simulink model "Antriebsstrangmodell_V1_4_n5"  (R2019a)
settings: Solver=FixedStepAuto  StartTime=0.0  StopTime=t_Simulation  FixedStep=dt  RelTol=1e-3
values from neighbouring files (symbols this model uses):
  A_Stirn = 2    [SIMULA~1.M]    (also in SIMULA~2.M)
  alpha_Luft = -4e-3    (= -0.004)    [SIMULA~1.M]    (also in SIMULA~2.M)
  alpha_Rotor = alpha_Al    (= 0.004)    [SIMULA~1.M]    (also in SIMULA~2.M)
  alpha_Stator = alpha_Al    (= 0.004)    [SIMULA~1.M]    (also in SIMULA~2.M)
  alpha_Ummag = -0.75e-3    (= -0.00075)    [SIMULA~1.M]    (also in SIMULA~2.M)
  c_W = 0.37    [SIMULA~1.M]    (also in SIMULA~2.M)
  COG_x = 1.4267    [SIMULA~1.M]    (also in SIMULA~2.M)
  COG_z = 0.4572    [SIMULA~1.M]    (also in SIMULA~2.M)
  cp_Luft = 1008.8    [SIMULA~1.M]    (also in SIMULA~2.M)
  e_Fahrzeug = 1.0478    [SIMULA~1.M]    (also in SIMULA~2.M)
  eta_EMaschine_Break_M_EMaschine = flipud(KennfeldMaschine.M(:,1))'    [SIMULA~1.M]    (also in SIMULA~2.M)
  eta_EMaschine_Break_M_EMaschine_reku = -KennfeldMaschine.M(:,1)'    [SIMULA~1.M]    (also in SIMULA~2.M)
  eta_EMaschine_Break_n_EMaschine = KennfeldMaschine.n(end-1,:)    [SIMULA~1.M]    (also in SIMULA~2.M)
  eta_EMaschine_Break_n_EMaschine_reku = KennfeldMaschine.n(end-1,:)    [SIMULA~1.M]    (also in SIMULA~2.M)
  eta_EMaschine_Faktor_Volllast = 0.98    [SIMULA~1.M]    (also in SIMULA~2.M)
  eta_EMaschine_Table = flip(KennfeldMaschine.etages,1)    [SIMULA~1.M]    (also in SIMULA~2.M)
  eta_EMaschine_Table_reku = KennfeldMaschine.etages    [SIMULA~1.M]    (also in SIMULA~2.M)
  eta_Getriebe = 0.96    [SIMULA~1.M]    (also in SIMULA~2.M)
  eta_IA = 0.5    [SIMULA~1.M]    (also in SIMULA~2.M)
  h_WC_pumpoff = Nu_WC*lam_WC/dh_WC    [SIMULA~1.M]    (also in SIMULA~2.M)
  h_WC_pumpon = Nu_WC*lam_WC/dh_WC    [SIMULA~1.M]    (also in SIMULA~2.M)
  i_Getriebe = 5.697    [SIMULA~1.M]    (also in SIMULA~2.M)
  krb_Korrektur = 0.53/10    (= 0.053)    [SIMULA~1.M]    (also in SIMULA~2.M)
  lam_Luft = 0.028592    [SIMULA~1.M]    (also in SIMULA~2.M)
  M_EMaschine_max = zeros(2,numel(eta_EMaschine_Break_n_EMaschine))    [SIMULA~1.M]    (also in SIMULA~2.M)
  m_Fahrzeug = 825    [SIMULA~1.M]    (also in SIMULA~2.M)
  m_Zuladung = 80    [SIMULA~1.M]    (also in SIMULA~2.M)
  nue_Luft = 19.230034390524e-6    (= 1.92300343905e-05)    [SIMULA~1.M]    (also in SIMULA~2.M)
  pump_start_limit = 273.15 + 33    (= 306.15)    [SIMULA~1.M]    (also in SIMULA~2.M)
  r_dynamisch = 0.2774    [SIMULA~1.M]    (also in SIMULA~2.M)
  rho_Luft = 1.2    [SIMULA~1.M]    (also in SIMULA~2.M)
  rho_Luft_EM = 1.0468    [SIMULA~1.M]    (also in SIMULA~2.M)
  share_EMaschine_Ummagnet_reku_Table = ser.gen.share_Ummagnetisierungsverluste    [SIMULA~1.M]    (also in SIMULA~2.M)
  share_EMaschine_Ummagnet_Table = ser.mot.share_Ummagnetisierungsverluste    [SIMULA~1.M]    (also in SIMULA~2.M)
  share_EMaschine_Wicklung_reku_Table = ser.gen.share_Wicklungsverluste    [SIMULA~1.M]    (also in SIMULA~2.M)
  share_EMaschine_Wicklung_Table = ser.mot.share_Wicklungsverluste    [SIMULA~1.M]    (also in SIMULA~2.M)
  share_EMaschine_WirkMech_reku_Table = ser.gen.share_WirkmechVerluste    [SIMULA~1.M]    (also in SIMULA~2.M)
  share_EMaschine_WirkMech_Table = ser.mot.share_WirkmechVerluste    [SIMULA~1.M]    (also in SIMULA~2.M)
  share_EMaschine_WirkZus_reku_Table = ser.gen.share_WirkZusVerl    [SIMULA~1.M]    (also in SIMULA~2.M)
  share_EMaschine_WirkZus_Table = ser.mot.share_WirkZusVerl    [SIMULA~1.M]    (also in SIMULA~2.M)
  T_Entwurf_Rotor = 273.15+20    (= 293.15)    [SIMULA~1.M]    (also in SIMULA~2.M)
  T_Entwurf_Stator = 273.15+20    (= 293.15)    [SIMULA~1.M]    (also in SIMULA~2.M)
  t_Simulation = v_Fahrzeug.Time(end)+1    [SIMULA~1.M]    (also in SIMULA~2.M = v_Fahrzeug.Time(end))
  T_Start_EMaschine = 273.15 + 23    (= 296.15)    [SIMULA~1.M]    (also in SIMULA~2.M)
  v_max = 110    [SIMULA~1.M]    (also in SIMULA~2.M)
  WB = 2.96    [SIMULA~1.M]    (also in SIMULA~2.M)
undefined symbols (not defined in the file or in its folder): A_AGP, A_IA, Anteil_Rotor_Ringe, Anteil_Stator, chi_Lager, D_2a, D_2r, delta, f_R, m_RTO, m_RYO, m_SSL_L, m_STO, m_SYO, m_WH_L, n_dis
libraries: fl_lib x440, nesl_utility x106, SimscapeCustomBlocks_lib x45, simulink x3
(part 2 of 5)

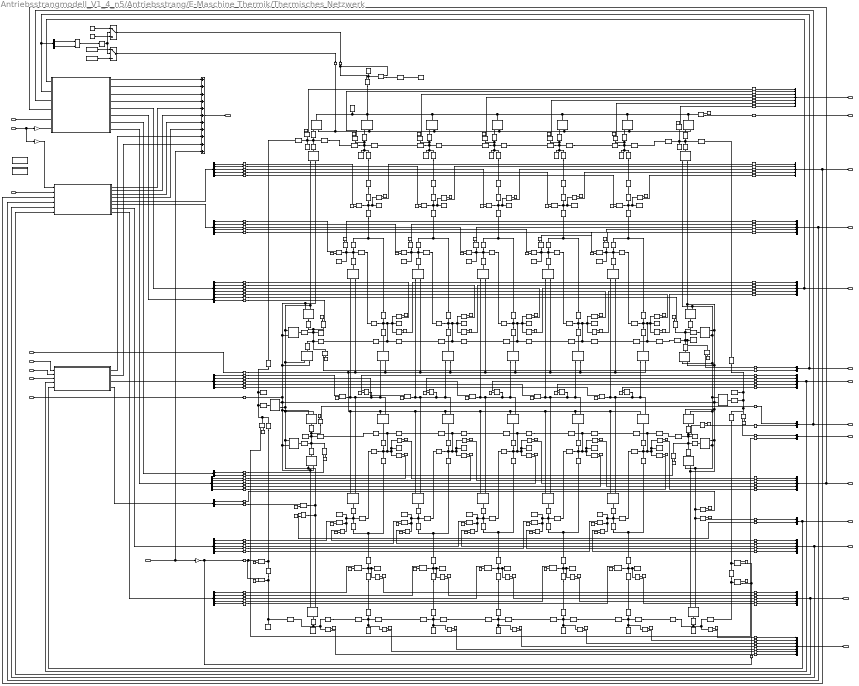
== system Antriebsstrangmodell_V1_4_n5/Antriebsstrang/E-Maschine Thermik/Thermisches Netzwerk ==
  note: Gehäusedeckel
  note: Gehäusedeckel
  note: Statorzähne
  note: Rotornuten
  note: Rotorwelle
  note: Lager
  note: Lager
  note: Rotorrücken
  note: Rotorzähne
  note: Kurzschluss-
      | ring
  note: Kurzschlussring
  note: Wickelkopf
  note: Wickelkopf
  note: Statornuten (Wicklung)
  note: Statorjoch
  note: Gehäuse
  P_EMaschine_Verlust_Wicklung [W] : Inport
  P_EMaschine_Verlust_Ummagnet [W] : Inport  Port=2
  P_EMaschine_Verlust_WirkZus [W] : Inport  Port=3
  P_EMaschine_Verlust_Lueftung [W] : Inport  Port=4
  P_EMaschine_Verlust_Lager [W] : Inport  Port=5
  HTC_Luftspalt [W*m^-2*K^-1] : Inport  Port=6
  HTC_fconv_Luftspalt [W*m^-2*K^-1] : Inport  Port=7
  HTC_Innenluft [W*m^-2*K^-1] : Inport  Port=8
  HTC_fconv_Innenluft [W*m^-2*K^-1] : Inport  Port=9
  Add : Sum  Inputs=+++++++++++
  Aufteilung + Temperaturabhängigkeit Lüftungsverluste : Subsystem
  Aufteilung + Temperaturabhängigkeit Ummagnetisierungsverluste : Subsystem
  Aufteilung Wicklungsverluste + Temperaturabhängiger ohmscher Widerstand : Subsystem
  Bus Creator{,1,3..7} (7 alike) : BusCreator  Inputs=5
  Bus Creator10 : BusCreator  Inputs=7
  Bus Creator11 : BusCreator  Inputs=7
  Bus Creator{2,8..9,12} (4 alike) : BusCreator  Inputs=2
  Bus Selector : BusSelector  OutputSignals=P_EMaschine_Verlust_SSL_1 [W],P_EMaschine_Verlust_SSL_2 [W],P_EMaschine_Verlust_SSL_3 [W],P_EMaschine_Verlust_SSL_4 [W],P_EMaschine_Verlust_SSL_5 [W]
  Bus Selector1 : BusSelector  OutputSignals=T_EMaschine_WH_2 [K],T_EMaschine_WH_1 [K]
  Bus Selector10 : BusSelector  OutputSignals=P_EMaschine_Verlust_IA_2 [W],P_EMaschine_Verlust_IA_1 [W]
  Bus Selector2 : BusSelector  OutputSignals=P_EMaschine_Verlust_WH_2 [W],P_EMaschine_Verlust_WH_1 [W]
  Bus Selector3 : BusSelector  OutputSignals=P_EMaschine_Verlust_ER_1 [W],P_EMaschine_Verlust_ER_2 [W]
  Bus Selector4 : BusSelector  OutputSignals=P_EMaschine_Verlust_RSL_1 [W],P_EMaschine_Verlust_RSL_2 [W],P_EMaschine_Verlust_RSL_3 [W],P_EMaschine_Verlust_RSL_4 [W],P_EMaschine_Verlust_RSL_5 [W]
  Bus Selector5 : BusSelector  OutputSignals=P_EMaschine_Verlust_AGP_1 [W],P_EMaschine_Verlust_AGP_2 [W],P_EMaschine_Verlust_AGP_3 [W],P_EMaschine_Verlust_AGP_4 [W],P_EMaschine_Verlust_AGP_5 [W]
  Bus Selector6 : BusSelector  OutputSignals=P_EMaschine_Verlust_STO_1 [W],P_EMaschine_Verlust_STO_2 [W],P_EMaschine_Verlust_STO_3 [W],P_EMaschine_Verlust_STO_4 [W],P_EMaschine_Verlust_STO_5 [W]
  Bus Selector7 : BusSelector  OutputSignals=P_EMaschine_Verlust_SYO_1 [W],P_EMaschine_Verlust_SYO_2 [W],P_EMaschine_Verlust_SYO_3 [W],P_EMaschine_Verlust_SYO_4 [W],P_EMaschine_Verlust_SYO_5 [W]
  Bus Selector8 : BusSelector  OutputSignals=P_EMaschine_Verlust_RTO_1 [W],P_EMaschine_Verlust_RTO_2 [W],P_EMaschine_Verlust_RTO_3 [W],P_EMaschine_Verlust_RTO_4 [W],P_EMaschine_Verlust_RTO_5 [W]
  Bus Selector9 : BusSelector  OutputSignals=P_EMaschine_Verlust_RYO_1 [W],P_EMaschine_Verlust_RYO_2 [W],P_EMaschine_Verlust_RYO_3 [W],P_EMaschine_Verlust_RYO_4 [W],P_EMaschine_Verlust_RYO_5 [W]
  C_EC(1) : fl_lib/Thermal/Thermal Elements/Thermal Mass  mass=m_EC kg  sp_heat=cp_EC J/kg/K  T_specify=on  T_priority=High  T=T_Start_EMaschine K  T_nominal_specify=off  T_nominal_unit=K  T_nominal_value=1  Q_specify=off  Q_priority=None  Q=0 W  Q_nominal_specify=off  Q_nominal_unit=W  Q_nominal_value=1
  C_EC(2) : fl_lib/Thermal/Thermal Elements/Thermal Mass  mass=m_EC kg  sp_heat=cp_EC J/kg/K  T_specify=on  T_priority=High  T=T_Start_EMaschine K  T_nominal_specify=off  T_nominal_unit=K  T_nominal_value=1  Q_specify=off  Q_priority=None  Q=0 W  Q_nominal_specify=off  Q_nominal_unit=W  Q_nominal_value=1
  C_ER(1) : fl_lib/Thermal/Thermal Elements/Thermal Mass  mass=m_ER kg  sp_heat=cp_ER J/kg/K  T_specify=on  T_priority=High  T=T_Start_EMaschine K  T_nominal_specify=off  T_nominal_unit=K  T_nominal_value=1  Q_specify=off  Q_priority=None  Q=0 W  Q_nominal_specify=off  Q_nominal_unit=W  Q_nominal_value=1
  C_ER(2) : fl_lib/Thermal/Thermal Elements/Thermal Mass  mass=m_ER kg  sp_heat=cp_ER J/kg/K  T_specify=on  T_priority=High  T=T_Start_EMaschine K  T_nominal_specify=off  T_nominal_unit=K  T_nominal_value=1  Q_specify=off  Q_priority=None  Q=0 W  Q_nominal_specify=off  Q_nominal_unit=W  Q_nominal_value=1
  C_HO_a(1) : fl_lib/Thermal/Thermal Elements/Thermal Mass  mass=m_HO_a kg  sp_heat=cp_HO J/kg/K  T_specify=on  T_priority=High  T=T_Start_EMaschine K  T_nominal_specify=off  T_nominal_unit=K  T_nominal_value=1  Q_specify=off  Q_priority=None  Q=0 W  Q_nominal_specify=off  Q_nominal_unit=W  Q_nominal_value=1
  C_HO_a(2) : fl_lib/Thermal/Thermal Elements/Thermal Mass  mass=m_HO_a kg  sp_heat=cp_HO J/kg/K  T_specify=on  T_priority=High  T=T_Start_EMaschine K  T_nominal_specify=off  T_nominal_unit=K  T_nominal_value=1  Q_specify=off  Q_priority=None  Q=0 W  Q_nominal_specify=off  Q_nominal_unit=W  Q_nominal_value=1
  C_HO_a(3) : fl_lib/Thermal/Thermal Elements/Thermal Mass  mass=m_HO_a kg  sp_heat=cp_HO J/kg/K  T_specify=on  T_priority=High  T=T_Start_EMaschine K  T_nominal_specify=off  T_nominal_unit=K  T_nominal_value=1  Q_specify=off  Q_priority=None  Q=0 W  Q_nominal_specify=off  Q_nominal_unit=W  Q_nominal_value=1
  C_HO_a(4) : fl_lib/Thermal/Thermal Elements/Thermal Mass  mass=m_HO_a kg  sp_heat=cp_HO J/kg/K  T_specify=on  T_priority=High  T=T_Start_EMaschine K  T_nominal_specify=off  T_nominal_unit=K  T_nominal_value=1  Q_specify=off  Q_priority=None  Q=0 W  Q_nominal_specify=off  Q_nominal_unit=W  Q_nominal_value=1
  C_HO_a(5) : fl_lib/Thermal/Thermal Elements/Thermal Mass  mass=m_HO_a kg  sp_heat=cp_HO J/kg/K  T_specify=on  T_priority=High  T=T_Start_EMaschine K  T_nominal_specify=off  T_nominal_unit=K  T_nominal_value=1  Q_specify=off  Q_priority=None  Q=0 W  Q_nominal_specify=off  Q_nominal_unit=W  Q_nominal_value=1
  C_HO_p(1) : fl_lib/Thermal/Thermal Elements/Thermal Mass  mass=m_HO_p kg  sp_heat=cp_HO J/kg/K  T_specify=on  T_priority=High  T=T_Start_EMaschine K  T_nominal_specify=off  T_nominal_unit=K  T_nominal_value=1  Q_specify=off  Q_priority=None  Q=0 W  Q_nominal_specify=off  Q_nominal_unit=W  Q_nominal_value=1
  C_HO_p(2) : fl_lib/Thermal/Thermal Elements/Thermal Mass  mass=m_HO_p kg  sp_heat=cp_HO J/kg/K  T_specify=on  T_priority=High  T=T_Start_EMaschine K  T_nominal_specify=off  T_nominal_unit=K  T_nominal_value=1  Q_specify=off  Q_priority=None  Q=0 W  Q_nominal_specify=off  Q_nominal_unit=W  Q_nominal_value=1
  C_RSL(1) : fl_lib/Thermal/Thermal Elements/Thermal Mass  mass=m_RSL kg  sp_heat=cp_RSL J/kg/K  T_specify=on  T_priority=High  T=T_Start_EMaschine K  T_nominal_specify=off  T_nominal_unit=K  T_nominal_value=1  Q_specify=off  Q_priority=None  Q=0 W  Q_nominal_specify=off  Q_nominal_unit=W  Q_nominal_value=1
  C_RSL(2) : fl_lib/Thermal/Thermal Elements/Thermal Mass  mass=m_RSL kg  sp_heat=cp_RSL J/kg/K  T_specify=on  T_priority=High  T=T_Start_EMaschine K  T_nominal_specify=off  T_nominal_unit=K  T_nominal_value=1  Q_specify=off  Q_priority=None  Q=0 W  Q_nominal_specify=off  Q_nominal_unit=W  Q_nominal_value=1
  C_RSL(3) : fl_lib/Thermal/Thermal Elements/Thermal Mass  mass=m_RSL kg  sp_heat=cp_RSL J/kg/K  T_specify=on  T_priority=High  T=T_Start_EMaschine K  T_nominal_specify=off  T_nominal_unit=K  T_nominal_value=1  Q_specify=off  Q_priority=None  Q=0 W  Q_nominal_specify=off  Q_nominal_unit=W  Q_nominal_value=1
  C_RSL(4) : fl_lib/Thermal/Thermal Elements/Thermal Mass  mass=m_RSL kg  sp_heat=cp_RSL J/kg/K  T_specify=on  T_priority=High  T=T_Start_EMaschine K  T_nominal_specify=off  T_nominal_unit=K  T_nominal_value=1  Q_specify=off  Q_priority=None  Q=0 W  Q_nominal_specify=off  Q_nominal_unit=W  Q_nominal_value=1
  C_RSL(5) : fl_lib/Thermal/Thermal Elements/Thermal Mass  mass=m_RSL kg  sp_heat=cp_RSL J/kg/K  T_specify=on  T_priority=High  T=T_Start_EMaschine K  T_nominal_specify=off  T_nominal_unit=K  T_nominal_value=1  Q_specify=off  Q_priority=None  Q=0 W  Q_nominal_specify=off  Q_nominal_unit=W  Q_nominal_value=1
  C_RTO(1) : fl_lib/Thermal/Thermal Elements/Thermal Mass  mass=m_RTO kg  sp_heat=cp_RTO J/kg/K  T_specify=on  T_priority=High  T=T_Start_EMaschine K  T_nominal_specify=off  T_nominal_unit=K  T_nominal_value=1  Q_specify=off  Q_priority=None  Q=0 W  Q_nominal_specify=off  Q_nominal_unit=W  Q_nominal_value=1
  C_RTO(2) : fl_lib/Thermal/Thermal Elements/Thermal Mass  mass=m_RTO kg  sp_heat=cp_RTO J/kg/K  T_specify=on  T_priority=High  T=T_Start_EMaschine K  T_nominal_specify=off  T_nominal_unit=K  T_nominal_value=1  Q_specify=off  Q_priority=None  Q=0 W  Q_nominal_specify=off  Q_nominal_unit=W  Q_nominal_value=1
  C_RTO(3) : fl_lib/Thermal/Thermal Elements/Thermal Mass  mass=m_RTO kg  sp_heat=cp_RTO J/kg/K  T_specify=on  T_priority=High  T=T_Start_EMaschine K  T_nominal_specify=off  T_nominal_unit=K  T_nominal_value=1  Q_specify=off  Q_priority=None  Q=0 W  Q_nominal_specify=off  Q_nominal_unit=W  Q_nominal_value=1
  C_RTO(4) : fl_lib/Thermal/Thermal Elements/Thermal Mass  mass=m_RTO kg  sp_heat=cp_RTO J/kg/K  T_specify=on  T_priority=High  T=T_Start_EMaschine K  T_nominal_specify=off  T_nominal_unit=K  T_nominal_value=1  Q_specify=off  Q_priority=None  Q=0 W  Q_nominal_specify=off  Q_nominal_unit=W  Q_nominal_value=1
  C_RTO(5) : fl_lib/Thermal/Thermal Elements/Thermal Mass  mass=m_RTO kg  sp_heat=cp_RTO J/kg/K  T_specify=on  T_priority=High  T=T_Start_EMaschine K  T_nominal_specify=off  T_nominal_unit=K  T_nominal_value=1  Q_specify=off  Q_priority=None  Q=0 W  Q_nominal_specify=off  Q_nominal_unit=W  Q_nominal_value=1
  C_RYO(1) : fl_lib/Thermal/Thermal Elements/Thermal Mass  mass=m_RYO kg  sp_heat=cp_RYO J/kg/K  T_specify=on  T_priority=High  T=T_Start_EMaschine K  T_nominal_specify=off  T_nominal_unit=K  T_nominal_value=1  Q_specify=off  Q_priority=None  Q=0 W  Q_nominal_specify=off  Q_nominal_unit=W  Q_nominal_value=1
  C_RYO(2) : fl_lib/Thermal/Thermal Elements/Thermal Mass  mass=m_RYO kg  sp_heat=cp_RYO J/kg/K  T_specify=on  T_priority=High  T=T_Start_EMaschine K  T_nominal_specify=off  T_nominal_unit=K  T_nominal_value=1  Q_specify=off  Q_priority=None  Q=0 W  Q_nominal_specify=off  Q_nominal_unit=W  Q_nominal_value=1
  C_RYO(3) : fl_lib/Thermal/Thermal Elements/Thermal Mass  mass=m_RYO kg  sp_heat=cp_RYO J/kg/K  T_specify=on  T_priority=High  T=T_Start_EMaschine K  T_nominal_specify=off  T_nominal_unit=K  T_nominal_value=1  Q_specify=off  Q_priority=None  Q=0 W  Q_nominal_specify=off  Q_nominal_unit=W  Q_nominal_value=1
  C_RYO(4) : fl_lib/Thermal/Thermal Elements/Thermal Mass  mass=m_RYO kg  sp_heat=cp_RYO J/kg/K  T_specify=on  T_priority=High  T=T_Start_EMaschine K  T_nominal_specify=off  T_nominal_unit=K  T_nominal_value=1  Q_specify=off  Q_priority=None  Q=0 W  Q_nominal_specify=off  Q_nominal_unit=W  Q_nominal_value=1
  C_RYO(5) : fl_lib/Thermal/Thermal Elements/Thermal Mass  mass=m_RYO kg  sp_heat=cp_RYO J/kg/K  T_specify=on  T_priority=High  T=T_Start_EMaschine K  T_nominal_specify=off  T_nominal_unit=K  T_nominal_value=1  Q_specify=off  Q_priority=None  Q=0 W  Q_nominal_specify=off  Q_nominal_unit=W  Q_nominal_value=1
  C_SH_a(1) : fl_lib/Thermal/Thermal Elements/Thermal Mass  mass=m_SH_a kg  sp_heat=cp_SH J/kg/K  T_specify=on  T_priority=High  T=T_Start_EMaschine K  T_nominal_specify=off  T_nominal_unit=K  T_nominal_value=1  Q_specify=off  Q_priority=None  Q=0 W  Q_nominal_specify=off  Q_nominal_unit=W  Q_nominal_value=1
  C_SH_a(2) : fl_lib/Thermal/Thermal Elements/Thermal Mass  mass=m_SH_a kg  sp_heat=cp_SH J/kg/K  T_specify=on  T_priority=High  T=T_Start_EMaschine K  T_nominal_specify=off  T_nominal_unit=K  T_nominal_value=1  Q_specify=off  Q_priority=None  Q=0 W  Q_nominal_specify=off  Q_nominal_unit=W  Q_nominal_value=1
  C_SH_a(3) : fl_lib/Thermal/Thermal Elements/Thermal Mass  mass=m_SH_a kg  sp_heat=cp_SH J/kg/K  T_specify=on  T_priority=High  T=T_Start_EMaschine K  T_nominal_specify=off  T_nominal_unit=K  T_nominal_value=1  Q_specify=off  Q_priority=None  Q=0 W  Q_nominal_specify=off  Q_nominal_unit=W  Q_nominal_value=1
  C_SH_a(4) : fl_lib/Thermal/Thermal Elements/Thermal Mass  mass=m_SH_a kg  sp_heat=cp_SH J/kg/K  T_specify=on  T_priority=High  T=T_Start_EMaschine K  T_nominal_specify=off  T_nominal_unit=K  T_nominal_value=1  Q_specify=off  Q_priority=None  Q=0 W  Q_nominal_specify=off  Q_nominal_unit=W  Q_nominal_value=1
  C_SH_a(5) : fl_lib/Thermal/Thermal Elements/Thermal Mass  mass=m_SH_a kg  sp_heat=cp_SH J/kg/K  T_specify=on  T_priority=High  T=T_Start_EMaschine K  T_nominal_specify=off  T_nominal_unit=K  T_nominal_value=1  Q_specify=off  Q_priority=None  Q=0 W  Q_nominal_specify=off  Q_nominal_unit=W  Q_nominal_value=1
  C_SH_p(1) : fl_lib/Thermal/Thermal Elements/Thermal Mass  mass=m_SH_p kg  sp_heat=cp_SH J/kg/K  T_specify=on  T_priority=High  T=T_Start_EMaschine K  T_nominal_specify=off  T_nominal_unit=K  T_nominal_value=1  Q_specify=off  Q_priority=None  Q=0 W  Q_nominal_specify=off  Q_nominal_unit=W  Q_nominal_value=1
  C_SH_p(2) : fl_lib/Thermal/Thermal Elements/Thermal Mass  mass=m_SH_p kg  sp_heat=cp_SH J/kg/K  T_specify=on  T_priority=High  T=T_Start_EMaschine K  T_nominal_specify=off  T_nominal_unit=K  T_nominal_value=1  Q_specify=off  Q_priority=None  Q=0 W  Q_nominal_specify=off  Q_nominal_unit=W  Q_nominal_value=1
  C_SSL(1) : fl_lib/Thermal/Thermal Elements/Thermal Mass  mass=m_SSL kg  sp_heat=cp_SSL J/kg/K  T_specify=on  T_priority=High  T=T_Start_EMaschine K  T_nominal_specify=off  T_nominal_unit=K  T_nominal_value=1  Q_specify=off  Q_priority=None  Q=0 W  Q_nominal_specify=off  Q_nominal_unit=W  Q_nominal_value=1
  C_SSL(2) : fl_lib/Thermal/Thermal Elements/Thermal Mass  mass=m_SSL kg  sp_heat=cp_SSL J/kg/K  T_specify=on  T_priority=High  T=T_Start_EMaschine K  T_nominal_specify=off  T_nominal_unit=K  T_nominal_value=1  Q_specify=off  Q_priority=None  Q=0 W  Q_nominal_specify=off  Q_nominal_unit=W  Q_nominal_value=1
  C_SSL(3) : fl_lib/Thermal/Thermal Elements/Thermal Mass  mass=m_SSL kg  sp_heat=cp_SSL J/kg/K  T_specify=on  T_priority=High  T=T_Start_EMaschine K  T_nominal_specify=off  T_nominal_unit=K  T_nominal_value=1  Q_specify=off  Q_priority=None  Q=0 W  Q_nominal_specify=off  Q_nominal_unit=W  Q_nominal_value=1
  C_SSL(4) : fl_lib/Thermal/Thermal Elements/Thermal Mass  mass=m_SSL kg  sp_heat=cp_SSL J/kg/K  T_specify=on  T_priority=High  T=T_Start_EMaschine K  T_nominal_specify=off  T_nominal_unit=K  T_nominal_value=1  Q_specify=off  Q_priority=None  Q=0 W  Q_nominal_specify=off  Q_nominal_unit=W  Q_nominal_value=1
  C_SSL(5) : fl_lib/Thermal/Thermal Elements/Thermal Mass  mass=m_SSL kg  sp_heat=cp_SSL J/kg/K  T_specify=on  T_priority=High  T=T_Start_EMaschine K  T_nominal_specify=off  T_nominal_unit=K  T_nominal_value=1  Q_specify=off  Q_priority=None  Q=0 W  Q_nominal_specify=off  Q_nominal_unit=W  Q_nominal_value=1
  C_STO(1) : fl_lib/Thermal/Thermal Elements/Thermal Mass  mass=m_STO kg  sp_heat=cp_STO J/kg/K  T_specify=on  T_priority=High  T=T_Start_EMaschine K  T_nominal_specify=off  T_nominal_unit=K  T_nominal_value=1  Q_specify=off  Q_priority=None  Q=0 W  Q_nominal_specify=off  Q_nominal_unit=W  Q_nominal_value=1
  C_STO(2) : fl_lib/Thermal/Thermal Elements/Thermal Mass  mass=m_STO kg  sp_heat=cp_STO J/kg/K  T_specify=on  T_priority=High  T=T_Start_EMaschine K  T_nominal_specify=off  T_nominal_unit=K  T_nominal_value=1  Q_specify=off  Q_priority=None  Q=0 W  Q_nominal_specify=off  Q_nominal_unit=W  Q_nominal_value=1
  C_STO(3) : fl_lib/Thermal/Thermal Elements/Thermal Mass  mass=m_STO kg  sp_heat=cp_STO J/kg/K  T_specify=on  T_priority=High  T=T_Start_EMaschine K  T_nominal_specify=off  T_nominal_unit=K  T_nominal_value=1  Q_specify=off  Q_priority=None  Q=0 W  Q_nominal_specify=off  Q_nominal_unit=W  Q_nominal_value=1
  C_STO(4) : fl_lib/Thermal/Thermal Elements/Thermal Mass  mass=m_STO kg  sp_heat=cp_STO J/kg/K  T_specify=on  T_priority=High  T=T_Start_EMaschine K  T_nominal_specify=off  T_nominal_unit=K  T_nominal_value=1  Q_specify=off  Q_priority=None  Q=0 W  Q_nominal_specify=off  Q_nominal_unit=W  Q_nominal_value=1
  C_STO(5) : fl_lib/Thermal/Thermal Elements/Thermal Mass  mass=m_STO kg  sp_heat=cp_STO J/kg/K  T_specify=on  T_priority=High  T=T_Start_EMaschine K  T_nominal_specify=off  T_nominal_unit=K  T_nominal_value=1  Q_specify=off  Q_priority=None  Q=0 W  Q_nominal_specify=off  Q_nominal_unit=W  Q_nominal_value=1
  C_SYO(1) : fl_lib/Thermal/Thermal Elements/Thermal Mass  mass=m_SYO kg  sp_heat=cp_SYO J/kg/K  T_specify=on  T_priority=High  T=T_Start_EMaschine K  T_nominal_specify=off  T_nominal_unit=K  T_nominal_value=1  Q_specify=off  Q_priority=None  Q=0 W  Q_nominal_specify=off  Q_nominal_unit=W  Q_nominal_value=1
  C_SYO(2) : fl_lib/Thermal/Thermal Elements/Thermal Mass  mass=m_SYO kg  sp_heat=cp_SYO J/kg/K  T_specify=on  T_priority=High  T=T_Start_EMaschine K  T_nominal_specify=off  T_nominal_unit=K  T_nominal_value=1  Q_specify=off  Q_priority=None  Q=0 W  Q_nominal_specify=off  Q_nominal_unit=W  Q_nominal_value=1
  C_SYO(3) : fl_lib/Thermal/Thermal Elements/Thermal Mass  mass=m_SYO kg  sp_heat=cp_SYO J/kg/K  T_specify=on  T_priority=High  T=T_Start_EMaschine K  T_nominal_specify=off  T_nominal_unit=K  T_nominal_value=1  Q_specify=off  Q_priority=None  Q=0 W  Q_nominal_specify=off  Q_nominal_unit=W  Q_nominal_value=1
  C_SYO(4) : fl_lib/Thermal/Thermal Elements/Thermal Mass  mass=m_SYO kg  sp_heat=cp_SYO J/kg/K  T_specify=on  T_priority=High  T=T_Start_EMaschine K  T_nominal_specify=off  T_nominal_unit=K  T_nominal_value=1  Q_specify=off  Q_priority=None  Q=0 W  Q_nominal_specify=off  Q_nominal_unit=W  Q_nominal_value=1
  C_SYO(5) : fl_lib/Thermal/Thermal Elements/Thermal Mass  mass=m_SYO kg  sp_heat=cp_SYO J/kg/K  T_specify=on  T_priority=High  T=T_Start_EMaschine K  T_nominal_specify=off  T_nominal_unit=K  T_nominal_value=1  Q_specify=off  Q_priority=None  Q=0 W  Q_nominal_specify=off  Q_nominal_unit=W  Q_nominal_value=1
  C_WC water cooling : fl_lib/Thermal/Thermal Elements/Thermal Mass  mass=m_WC kg  sp_heat=cp_WC J/kg/K  T_specify=on  T_priority=High  T=T_Start_EMaschine K  T_nominal_specify=off  T_nominal_unit=K  T_nominal_value=1  Q_specify=off  Q_priority=None  Q=0 W  Q_nominal_specify=off  Q_nominal_unit=W  Q_nominal_value=1
  C_WC water cooling pump active : fl_lib/Thermal/Thermal Elements/Thermal Mass  mass=m_WC_pumpon kg  sp_heat=cp_WC J/kg/K  T_specify=on  T_priority=High  T=T_Start_EMaschine K  T_nominal_specify=off  T_nominal_unit=K  T_nominal_value=1  Q_specify=off  Q_priority=None  Q=0 W  Q_nominal_specify=off  Q_nominal_unit=W  Q_nominal_value=1
  C_WH(1) : fl_lib/Thermal/Thermal Elements/Thermal Mass  mass=m_WH kg  sp_heat=cp_WH J/kg/K  T_specify=on  T_priority=High  T=T_Start_EMaschine K  T_nominal_specify=off  T_nominal_unit=K  T_nominal_value=1  Q_specify=off  Q_priority=None  Q=0 W  Q_nominal_specify=off  Q_nominal_unit=W  Q_nominal_value=1
  C_WH(2) : fl_lib/Thermal/Thermal Elements/Thermal Mass  mass=m_WH kg  sp_heat=cp_WH J/kg/K  T_specify=on  T_priority=High  T=T_Start_EMaschine K  T_nominal_specify=off  T_nominal_unit=K  T_nominal_value=1  Q_specify=off  Q_priority=None  Q=0 W  Q_nominal_specify=off  Q_nominal_unit=W  Q_nominal_value=1
  Convection HO to coolant (1) : SimscapeCustomBlocks_lib/Convective Heat Transfer  area=A_HO_p m^2  T_specify=off  T_priority=None  T=0 K  T_nominal_specify=off  T_nominal_unit=K  T_nominal_value=1  Q_specify=off  Q_priority=None  Q=0 W  Q_nominal_specify=off  Q_nominal_unit=W  Q_nominal_value=1
  Convection HO to coolant (2) : SimscapeCustomBlocks_lib/Convective Heat Transfer  area=A_HO_a m^2  T_specify=off  T_priority=None  T=0 K  T_nominal_specify=off  T_nominal_unit=K  T_nominal_value=1  Q_specify=off  Q_priority=None  Q=0 W  Q_nominal_specify=off  Q_nominal_unit=W  Q_nominal_value=1
  Convection HO to coolant (3) : SimscapeCustomBlocks_lib/Convective Heat Transfer  area=A_HO_a m^2  T_specify=off  T_priority=None  T=0 K  T_nominal_specify=off  T_nominal_unit=K  T_nominal_value=1  Q_specify=off  Q_priority=None  Q=0 W  Q_nominal_specify=off  Q_nominal_unit=W  Q_nominal_value=1
  Convection HO to coolant (4) : SimscapeCustomBlocks_lib/Convective Heat Transfer  area=A_HO_a m^2  T_specify=off  T_priority=None  T=0 K  T_nominal_specify=off  T_nominal_unit=K  T_nominal_value=1  Q_specify=off  Q_priority=None  Q=0 W  Q_nominal_specify=off  Q_nominal_unit=W  Q_nominal_value=1
  Convection HO to coolant (5) : SimscapeCustomBlocks_lib/Convective Heat Transfer  area=A_HO_a m^2  T_specify=off  T_priority=None  T=0 K  T_nominal_specify=off  T_nominal_unit=K  T_nominal_value=1  Q_specify=off  Q_priority=None  Q=0 W  Q_nominal_specify=off  Q_nominal_unit=W  Q_nominal_value=1
  Convection HO to coolant (6) : SimscapeCustomBlocks_lib/Convective Heat Transfer  area=A_HO_a m^2  T_specify=off  T_priority=None  T=0 K  T_nominal_specify=off  T_nominal_unit=K  T_nominal_value=1  Q_specify=off  Q_priority=None  Q=0 W  Q_nominal_specify=off  Q_nominal_unit=W  Q_nominal_value=1
  Convection HO to coolant (7) : SimscapeCustomBlocks_lib/Convective Heat Transfer  area=A_HO_p m^2  T_specify=off  T_priority=None  T=0 K  T_nominal_specify=off  T_nominal_unit=K  T_nominal_value=1  Q_specify=off  Q_priority=None  Q=0 W  Q_nominal_specify=off  Q_nominal_unit=W  Q_nominal_value=1
  Delay : Delay
  Gain4 : Gain  Gain=1/4
  HTC with coolant pump active : Constant  Value=h_WC_pumpon
  HTC with coolant pump inactive : Constant  Value=h_WC_pumpoff
  Konvektion Radiator an Umgebungsluft (keine Geschw.Abhängigkeit) : fl_lib/Thermal/Thermal Elements/Convective Heat Transfer  area=1 m^2  heat_tr_coeff=radiator_power W/(m^2 * K)  T_specify=off  T_priority=None  T=0 K  T_nominal_specify=off  T_nominal_unit=K  T_nominal_value=1  Q_specify=off  Q_priority=None  Q=0 W  Q_nominal_specify=off  Q_nominal_unit=W  Q_nominal_value=1
  MinMax : MinMax  Function=max  Inputs=2
  PS-Simulink Converter{1..58} (58 alike) : nesl_utility/PS-Simulink Converter  PhysicalDomain=network_engine_domain  SubClassName=ps_output  LeftPortType=input  RightPortType=output  PseudoPeriodic=off  Frequencies=[]  Unit=1  AffineConversion=off
  PV_AGP(1) : fl_lib/Thermal/Thermal Sources/Controlled Heat Flow Rate Source
      settings: SourceProductName=Simscape
  PV_AGP(2) : fl_lib/Thermal/Thermal Sources/Controlled Heat Flow Rate Source
      settings: SourceProductName=Simscape
  PV_AGP(3) : fl_lib/Thermal/Thermal Sources/Controlled Heat Flow Rate Source
      settings: SourceProductName=Simscape
  PV_AGP(4) : fl_lib/Thermal/Thermal Sources/Controlled Heat Flow Rate Source
      settings: SourceProductName=Simscape
  PV_AGP(5) : fl_lib/Thermal/Thermal Sources/Controlled Heat Flow Rate Source
      settings: SourceProductName=Simscape
  PV_BR(1.1) : fl_lib/Thermal/Thermal Sources/Controlled Heat Flow Rate Source
      settings: SourceProductName=Simscape
  PV_BR(1.2) : fl_lib/Thermal/Thermal Sources/Controlled Heat Flow Rate Source
      settings: SourceProductName=Simscape
  PV_BR(2.1) : fl_lib/Thermal/Thermal Sources/Controlled Heat Flow Rate Source
      settings: SourceProductName=Simscape
  PV_BR(2.2) : fl_lib/Thermal/Thermal Sources/Controlled Heat Flow Rate Source
      settings: SourceProductName=Simscape
  PV_ER(1) : fl_lib/Thermal/Thermal Sources/Controlled Heat Flow Rate Source
      settings: SourceProductName=Simscape
  PV_ER(2) : fl_lib/Thermal/Thermal Sources/Controlled Heat Flow Rate Source
      settings: SourceProductName=Simscape
  PV_IA(1) : fl_lib/Thermal/Thermal Sources/Controlled Heat Flow Rate Source
      settings: SourceProductName=Simscape
  PV_IA(2) : fl_lib/Thermal/Thermal Sources/Controlled Heat Flow Rate Source
      settings: SourceProductName=Simscape
  PV_RSL(1) : fl_lib/Thermal/Thermal Sources/Controlled Heat Flow Rate Source
      settings: SourceProductName=Simscape
  PV_RSL(2) : fl_lib/Thermal/Thermal Sources/Controlled Heat Flow Rate Source
      settings: SourceProductName=Simscape
  PV_RSL(3) : fl_lib/Thermal/Thermal Sources/Controlled Heat Flow Rate Source
      settings: SourceProductName=Simscape
  PV_RSL(4) : fl_lib/Thermal/Thermal Sources/Controlled Heat Flow Rate Source
      settings: SourceProductName=Simscape
  PV_RSL(5) : fl_lib/Thermal/Thermal Sources/Controlled Heat Flow Rate Source
      settings: SourceProductName=Simscape
  PV_RTO(1) : fl_lib/Thermal/Thermal Sources/Controlled Heat Flow Rate Source
      settings: SourceProductName=Simscape
  PV_RTO(2) : fl_lib/Thermal/Thermal Sources/Controlled Heat Flow Rate Source
      settings: SourceProductName=Simscape
  PV_RTO(3) : fl_lib/Thermal/Thermal Sources/Controlled Heat Flow Rate Source
      settings: SourceProductName=Simscape
  PV_RTO(4) : fl_lib/Thermal/Thermal Sources/Controlled Heat Flow Rate Source
      settings: SourceProductName=Simscape
  PV_RTO(5) : fl_lib/Thermal/Thermal Sources/Controlled Heat Flow Rate Source
      settings: SourceProductName=Simscape
  PV_RYO(1) : fl_lib/Thermal/Thermal Sources/Controlled Heat Flow Rate Source
      settings: SourceProductName=Simscape
  PV_RYO(2) : fl_lib/Thermal/Thermal Sources/Controlled Heat Flow Rate Source
      settings: SourceProductName=Simscape
  PV_RYO(3) : fl_lib/Thermal/Thermal Sources/Controlled Heat Flow Rate Source
      settings: SourceProductName=Simscape
  PV_RYO(4) : fl_lib/Thermal/Thermal Sources/Controlled Heat Flow Rate Source
      settings: SourceProductName=Simscape
  PV_RYO(5) : fl_lib/Thermal/Thermal Sources/Controlled Heat Flow Rate Source
      settings: SourceProductName=Simscape
  PV_SSL(1) : fl_lib/Thermal/Thermal Sources/Controlled Heat Flow Rate Source
      settings: SourceProductName=Simscape
  PV_SSL(2) : fl_lib/Thermal/Thermal Sources/Controlled Heat Flow Rate Source
      settings: SourceProductName=Simscape
  PV_SSL(3) : fl_lib/Thermal/Thermal Sources/Controlled Heat Flow Rate Source
      settings: SourceProductName=Simscape
  PV_SSL(4) : fl_lib/Thermal/Thermal Sources/Controlled Heat Flow Rate Source
      settings: SourceProductName=Simscape
  PV_SSL(5) : fl_lib/Thermal/Thermal Sources/Controlled Heat Flow Rate Source
      settings: SourceProductName=Simscape
  PV_STO(1) : fl_lib/Thermal/Thermal Sources/Controlled Heat Flow Rate Source
      settings: SourceProductName=Simscape
  PV_STO(2) : fl_lib/Thermal/Thermal Sources/Controlled Heat Flow Rate Source
      settings: SourceProductName=Simscape
  PV_STO(3) : fl_lib/Thermal/Thermal Sources/Controlled Heat Flow Rate Source
      settings: SourceProductName=Simscape
  PV_STO(4) : fl_lib/Thermal/Thermal Sources/Controlled Heat Flow Rate Source
      settings: SourceProductName=Simscape
  PV_STO(5) : fl_lib/Thermal/Thermal Sources/Controlled Heat Flow Rate Source
      settings: SourceProductName=Simscape
  PV_SYO(1) : fl_lib/Thermal/Thermal Sources/Controlled Heat Flow Rate Source
      settings: SourceProductName=Simscape
  PV_SYO(2) : fl_lib/Thermal/Thermal Sources/Controlled Heat Flow Rate Source
      settings: SourceProductName=Simscape
  PV_SYO(3) : fl_lib/Thermal/Thermal Sources/Controlled Heat Flow Rate Source
      settings: SourceProductName=Simscape
  PV_SYO(4) : fl_lib/Thermal/Thermal Sources/Controlled Heat Flow Rate Source
      settings: SourceProductName=Simscape
  PV_SYO(5) : fl_lib/Thermal/Thermal Sources/Controlled Heat Flow Rate Source
      settings: SourceProductName=Simscape
  PV_WH(1) : fl_lib/Thermal/Thermal Sources/Controlled Heat Flow Rate Source
      settings: SourceProductName=Simscape
  PV_WH(2) : fl_lib/Thermal/Thermal Sources/Controlled Heat Flow Rate Source
      settings: SourceProductName=Simscape
  R_contactBR(1) : fl_lib/Thermal/Thermal Elements/Thermal Resistance  resistance=R_contactBR K/W  T_specify=off  T_priority=None  T=0 K  T_nominal_specify=off  T_nominal_unit=K  T_nominal_value=1  Q_specify=off  Q_priority=None  Q=0 W  Q_nominal_specify=off  Q_nominal_unit=W  Q_nominal_value=1
      settings: SourceProductName=Simscape  SourceProductBaseCode=SS
  R_contactBR(2) : fl_lib/Thermal/Thermal Elements/Thermal Resistance  resistance=R_contactBR K/W  T_specify=off  T_priority=None  T=0 K  T_nominal_specify=off  T_nominal_unit=K  T_nominal_value=1  Q_specify=off  Q_priority=None  Q=0 W  Q_nominal_specify=off  Q_nominal_unit=W  Q_nominal_value=1
      settings: SourceProductName=Simscape  SourceProductBaseCode=SS
  R_contactHO (1) : fl_lib/Thermal/Thermal Elements/Thermal Resistance  resistance=R_contactHO K/W  T_specify=off  T_priority=None  T=0 K  T_nominal_specify=off  T_nominal_unit=K  T_nominal_value=1  Q_specify=off  Q_priority=None  Q=0 W  Q_nominal_specify=off  Q_nominal_unit=W  Q_nominal_value=1
      settings: SourceProductName=Simscape  SourceProductBaseCode=SS
  R_contactHO (2) : fl_lib/Thermal/Thermal Elements/Thermal Resistance  resistance=R_contactHO K/W  T_specify=off  T_priority=None  T=0 K  T_nominal_specify=off  T_nominal_unit=K  T_nominal_value=1  Q_specify=off  Q_priority=None  Q=0 W  Q_nominal_specify=off  Q_nominal_unit=W  Q_nominal_value=1
      settings: SourceProductName=Simscape  SourceProductBaseCode=SS
  R_contactHO (3) : fl_lib/Thermal/Thermal Elements/Thermal Resistance  resistance=R_contactHO K/W  T_specify=off  T_priority=None  T=0 K  T_nominal_specify=off  T_nominal_unit=K  T_nominal_value=1  Q_specify=off  Q_priority=None  Q=0 W  Q_nominal_specify=off  Q_nominal_unit=W  Q_nominal_value=1
      settings: SourceProductName=Simscape  SourceProductBaseCode=SS
  R_contactHO (4) : fl_lib/Thermal/Thermal Elements/Thermal Resistance  resistance=R_contactHO K/W  T_specify=off  T_priority=None  T=0 K  T_nominal_specify=off  T_nominal_unit=K  T_nominal_value=1  Q_specify=off  Q_priority=None  Q=0 W  Q_nominal_specify=off  Q_nominal_unit=W  Q_nominal_value=1
      settings: SourceProductName=Simscape  SourceProductBaseCode=SS
  R_contactHO (5) : fl_lib/Thermal/Thermal Elements/Thermal Resistance  resistance=R_contactHO K/W  T_specify=off  T_priority=None  T=0 K  T_nominal_specify=off  T_nominal_unit=K  T_nominal_value=1  Q_specify=off  Q_priority=None  Q=0 W  Q_nominal_specify=off  Q_nominal_unit=W  Q_nominal_value=1
      settings: SourceProductName=Simscape  SourceProductBaseCode=SS
  R_toBR2(1) : fl_lib/Thermal/Thermal Elements/Thermal Resistance  resistance=R_toBR2 K/W  T_specify=off  T_priority=None  T=0 K  T_nominal_specify=off  T_nominal_unit=K  T_nominal_value=1  Q_specify=off  Q_priority=None  Q=0 W  Q_nominal_specify=off  Q_nominal_unit=W  Q_nominal_value=1
      settings: SourceProductName=Simscape  SourceProductBaseCode=SS
  R_toBR2(2) : fl_lib/Thermal/Thermal Elements/Thermal Resistance  resistance=R_toBR2 K/W  T_specify=off  T_priority=None  T=0 K  T_nominal_specify=off  T_nominal_unit=K  T_nominal_value=1  Q_specify=off  Q_priority=None  Q=0 W  Q_nominal_specify=off  Q_nominal_unit=W  Q_nominal_value=1
      settings: SourceProductName=Simscape  SourceProductBaseCode=SS
  R_toBR_a(1.1) : fl_lib/Thermal/Thermal Elements/Thermal Resistance  resistance=R_toBR_a K/W  T_specify=off  T_priority=None  T=0 K  T_nominal_specify=off  T_nominal_unit=K  T_nominal_value=1  Q_specify=off  Q_priority=None  Q=0 W  Q_nominal_specify=off  Q_nominal_unit=W  Q_nominal_value=1
      settings: SourceProductName=Simscape  SourceProductBaseCode=SS
  R_toBR_a(1.2) : fl_lib/Thermal/Thermal Elements/Thermal Resistance  resistance=R_toBR_a K/W  T_specify=off  T_priority=None  T=0 K  T_nominal_specify=off  T_nominal_unit=K  T_nominal_value=1  Q_specify=off  Q_priority=None  Q=0 W  Q_nominal_specify=off  Q_nominal_unit=W  Q_nominal_value=1
      settings: SourceProductName=Simscape  SourceProductBaseCode=SS
  R_toBR_a(2.1) : fl_lib/Thermal/Thermal Elements/Thermal Resistance  resistance=R_toBR_a K/W  T_specify=off  T_priority=None  T=0 K  T_nominal_specify=off  T_nominal_unit=K  T_nominal_value=1  Q_specify=off  Q_priority=None  Q=0 W  Q_nominal_specify=off  Q_nominal_unit=W  Q_nominal_value=1
      settings: SourceProductName=Simscape  SourceProductBaseCode=SS
  R_toBR_a(2.2) : fl_lib/Thermal/Thermal Elements/Thermal Resistance  resistance=R_toBR_a K/W  T_specify=off  T_priority=None  T=0 K  T_nominal_specify=off  T_nominal_unit=K  T_nominal_value=1  Q_specify=off  Q_priority=None  Q=0 W  Q_nominal_specify=off  Q_nominal_unit=W  Q_nominal_value=1
      settings: SourceProductName=Simscape  SourceProductBaseCode=SS
  R_toBR_a(3.1) : fl_lib/Thermal/Thermal Elements/Thermal Resistance  resistance=R_toBR_a K/W  T_specify=off  T_priority=None  T=0 K  T_nominal_specify=off  T_nominal_unit=K  T_nominal_value=1  Q_specify=off  Q_priority=None  Q=0 W  Q_nominal_specify=off  Q_nominal_unit=W  Q_nominal_value=1
      settings: SourceProductName=Simscape  SourceProductBaseCode=SS
  R_toBR_a(3.2) : fl_lib/Thermal/Thermal Elements/Thermal Resistance  resistance=R_toBR_a K/W  T_specify=off  T_priority=None  T=0 K  T_nominal_specify=off  T_nominal_unit=K  T_nominal_value=1  Q_specify=off  Q_priority=None  Q=0 W  Q_nominal_specify=off  Q_nominal_unit=W  Q_nominal_value=1
      settings: SourceProductName=Simscape  SourceProductBaseCode=SS
  R_toBR_a(4.1) : fl_lib/Thermal/Thermal Elements/Thermal Resistance  resistance=R_toBR_a K/W  T_specify=off  T_priority=None  T=0 K  T_nominal_specify=off  T_nominal_unit=K  T_nominal_value=1  Q_specify=off  Q_priority=None  Q=0 W  Q_nominal_specify=off  Q_nominal_unit=W  Q_nominal_value=1
      settings: SourceProductName=Simscape  SourceProductBaseCode=SS
  R_toBR_a(4.2) : fl_lib/Thermal/Thermal Elements/Thermal Resistance  resistance=R_toBR_a K/W  T_specify=off  T_priority=None  T=0 K  T_nominal_specify=off  T_nominal_unit=K  T_nominal_value=1  Q_specify=off  Q_priority=None  Q=0 W  Q_nominal_specify=off  Q_nominal_unit=W  Q_nominal_value=1
      settings: SourceProductName=Simscape  SourceProductBaseCode=SS
  R_toBR_a(5.1) : fl_lib/Thermal/Thermal Elements/Thermal Resistance  resistance=R_toBR_a K/W  T_specify=off  T_priority=None  T=0 K  T_nominal_specify=off  T_nominal_unit=K  T_nominal_value=1  Q_specify=off  Q_priority=None  Q=0 W  Q_nominal_specify=off  Q_nominal_unit=W  Q_nominal_value=1
      settings: SourceProductName=Simscape  SourceProductBaseCode=SS
  R_toBR_a(5.2) : fl_lib/Thermal/Thermal Elements/Thermal Resistance  resistance=R_toBR_a K/W  T_specify=off  T_priority=None  T=0 K  T_nominal_specify=off  T_nominal_unit=K  T_nominal_value=1  Q_specify=off  Q_priority=None  Q=0 W  Q_nominal_specify=off  Q_nominal_unit=W  Q_nominal_value=1
      settings: SourceProductName=Simscape  SourceProductBaseCode=SS
  R_toBR_p(1.1) : fl_lib/Thermal/Thermal Elements/Thermal Resistance  resistance=R_toBR_p K/W  T_specify=off  T_priority=None  T=0 K  T_nominal_specify=off  T_nominal_unit=K  T_nominal_value=1  Q_specify=off  Q_priority=None  Q=0 W  Q_nominal_specify=off  Q_nominal_unit=W  Q_nominal_value=1
      settings: SourceProductName=Simscape  SourceProductBaseCode=SS
  R_toBR_p(1.2) : fl_lib/Thermal/Thermal Elements/Thermal Resistance  resistance=R_toBR_p K/W  T_specify=off  T_priority=None  T=0 K  T_nominal_specify=off  T_nominal_unit=K  T_nominal_value=1  Q_specify=off  Q_priority=None  Q=0 W  Q_nominal_specify=off  Q_nominal_unit=W  Q_nominal_value=1
      settings: SourceProductName=Simscape  SourceProductBaseCode=SS
  R_toBR_p(2.1) : fl_lib/Thermal/Thermal Elements/Thermal Resistance  resistance=R_toBR_p K/W  T_specify=off  T_priority=None  T=0 K  T_nominal_specify=off  T_nominal_unit=K  T_nominal_value=1  Q_specify=off  Q_priority=None  Q=0 W  Q_nominal_specify=off  Q_nominal_unit=W  Q_nominal_value=1
      settings: SourceProductName=Simscape  SourceProductBaseCode=SS
  R_toBR_p(2.2) : fl_lib/Thermal/Thermal Elements/Thermal Resistance  resistance=R_toBR_p K/W  T_specify=off  T_priority=None  T=0 K  T_nominal_specify=off  T_nominal_unit=K  T_nominal_value=1  Q_specify=off  Q_priority=None  Q=0 W  Q_nominal_specify=off  Q_nominal_unit=W  Q_nominal_value=1
      settings: SourceProductName=Simscape  SourceProductBaseCode=SS
  R_toEC_a(1.1) : fl_lib/Thermal/Thermal Elements/Thermal Resistance  resistance=R_toEC_a K/W  T_specify=off  T_priority=None  T=0 K  T_nominal_specify=off  T_nominal_unit=K  T_nominal_value=1  Q_specify=off  Q_priority=None  Q=0 W  Q_nominal_specify=off  Q_nominal_unit=W  Q_nominal_value=1
      settings: SourceProductName=Simscape  SourceProductBaseCode=SS
  R_toEC_a(1.2) : fl_lib/Thermal/Thermal Elements/Thermal Resistance  resistance=R_toEC_a K/W  T_specify=off  T_priority=None  T=0 K  T_nominal_specify=off  T_nominal_unit=K  T_nominal_value=1  Q_specify=off  Q_priority=None  Q=0 W  Q_nominal_specify=off  Q_nominal_unit=W  Q_nominal_value=1
      settings: SourceProductName=Simscape  SourceProductBaseCode=SS
  R_toEC_a(2.1) : fl_lib/Thermal/Thermal Elements/Thermal Resistance  resistance=R_toEC_a K/W  T_specify=off  T_priority=None  T=0 K  T_nominal_specify=off  T_nominal_unit=K  T_nominal_value=1  Q_specify=off  Q_priority=None  Q=0 W  Q_nominal_specify=off  Q_nominal_unit=W  Q_nominal_value=1
      settings: SourceProductName=Simscape  SourceProductBaseCode=SS
  R_toEC_a(2.2) : fl_lib/Thermal/Thermal Elements/Thermal Resistance  resistance=R_toEC_a K/W  T_specify=off  T_priority=None  T=0 K  T_nominal_specify=off  T_nominal_unit=K  T_nominal_value=1  Q_specify=off  Q_priority=None  Q=0 W  Q_nominal_specify=off  Q_nominal_unit=W  Q_nominal_value=1
      settings: SourceProductName=Simscape  SourceProductBaseCode=SS
  R_toEC_a(3.1) : fl_lib/Thermal/Thermal Elements/Thermal Resistance  resistance=R_toEC_a K/W  T_specify=off  T_priority=None  T=0 K  T_nominal_specify=off  T_nominal_unit=K  T_nominal_value=1  Q_specify=off  Q_priority=None  Q=0 W  Q_nominal_specify=off  Q_nominal_unit=W  Q_nominal_value=1
      settings: SourceProductName=Simscape  SourceProductBaseCode=SS
  R_toEC_a(3.2) : fl_lib/Thermal/Thermal Elements/Thermal Resistance  resistance=R_toEC_a K/W  T_specify=off  T_priority=None  T=0 K  T_nominal_specify=off  T_nominal_unit=K  T_nominal_value=1  Q_specify=off  Q_priority=None  Q=0 W  Q_nominal_specify=off  Q_nominal_unit=W  Q_nominal_value=1
      settings: SourceProductName=Simscape  SourceProductBaseCode=SS
  R_toEC_a(4.1) : fl_lib/Thermal/Thermal Elements/Thermal Resistance  resistance=R_toEC_a K/W  T_specify=off  T_priority=None  T=0 K  T_nominal_specify=off  T_nominal_unit=K  T_nominal_value=1  Q_specify=off  Q_priority=None  Q=0 W  Q_nominal_specify=off  Q_nominal_unit=W  Q_nominal_value=1
      settings: SourceProductName=Simscape  SourceProductBaseCode=SS
  R_toEC_a(4.2) : fl_lib/Thermal/Thermal Elements/Thermal Resistance  resistance=R_toEC_a K/W  T_specify=off  T_priority=None  T=0 K  T_nominal_specify=off  T_nominal_unit=K  T_nominal_value=1  Q_specify=off  Q_priority=None  Q=0 W  Q_nominal_specify=off  Q_nominal_unit=W  Q_nominal_value=1
      settings: SourceProductName=Simscape  SourceProductBaseCode=SS
  R_toEC_a(5.1) : fl_lib/Thermal/Thermal Elements/Thermal Resistance  resistance=R_toEC_a K/W  T_specify=off  T_priority=None  T=0 K  T_nominal_specify=off  T_nominal_unit=K  T_nominal_value=1  Q_specify=off  Q_priority=None  Q=0 W  Q_nominal_specify=off  Q_nominal_unit=W  Q_nominal_value=1
      settings: SourceProductName=Simscape  SourceProductBaseCode=SS
  R_toEC_a(5.2) : fl_lib/Thermal/Thermal Elements/Thermal Resistance  resistance=R_toEC_a K/W  T_specify=off  T_priority=None  T=0 K  T_nominal_specify=off  T_nominal_unit=K  T_nominal_value=1  Q_specify=off  Q_priority=None  Q=0 W  Q_nominal_specify=off  Q_nominal_unit=W  Q_nominal_value=1
      settings: SourceProductName=Simscape  SourceProductBaseCode=SS
  R_toEC_p(1.1) : fl_lib/Thermal/Thermal Elements/Thermal Resistance  resistance=R_toEC_p K/W  T_specify=off  T_priority=None  T=0 K  T_nominal_specify=off  T_nominal_unit=K  T_nominal_value=1  Q_specify=off  Q_priority=None  Q=0 W  Q_nominal_specify=off  Q_nominal_unit=W  Q_nominal_value=1
      settings: SourceProductName=Simscape  SourceProductBaseCode=SS
  R_toEC_p(1.2) : fl_lib/Thermal/Thermal Elements/Thermal Resistance  resistance=R_toEC_p K/W  T_specify=off  T_priority=None  T=0 K  T_nominal_specify=off  T_nominal_unit=K  T_nominal_value=1  Q_specify=off  Q_priority=None  Q=0 W  Q_nominal_specify=off  Q_nominal_unit=W  Q_nominal_value=1
      settings: SourceProductName=Simscape  SourceProductBaseCode=SS
  R_toEC_p(2.1) : fl_lib/Thermal/Thermal Elements/Thermal Resistance  resistance=R_toEC_p K/W  T_specify=off  T_priority=None  T=0 K  T_nominal_specify=off  T_nominal_unit=K  T_nominal_value=1  Q_specify=off  Q_priority=None  Q=0 W  Q_nominal_specify=off  Q_nominal_unit=W  Q_nominal_value=1
      settings: SourceProductName=Simscape  SourceProductBaseCode=SS
  R_toEC_p(2.2) : fl_lib/Thermal/Thermal Elements/Thermal Resistance  resistance=R_toEC_p K/W  T_specify=off  T_priority=None  T=0 K  T_nominal_specify=off  T_nominal_unit=K  T_nominal_value=1  Q_specify=off  Q_priority=None  Q=0 W  Q_nominal_specify=off  Q_nominal_unit=W  Q_nominal_value=1
      settings: SourceProductName=Simscape  SourceProductBaseCode=SS
  R_toER(1.1) : fl_lib/Thermal/Thermal Elements/Thermal Resistance  resistance=R_toER K/W  T_specify=off  T_priority=None  T=0 K  T_nominal_specify=off  T_nominal_unit=K  T_nominal_value=1  Q_specify=off  Q_priority=None  Q=0 W  Q_nominal_specify=off  Q_nominal_unit=W  Q_nominal_value=1
      settings: SourceProductName=Simscape  SourceProductBaseCode=SS
  R_toER(1.2) : fl_lib/Thermal/Thermal Elements/Thermal Resistance  resistance=R_toER K/W  T_specify=off  T_priority=None  T=0 K  T_nominal_specify=off  T_nominal_unit=K  T_nominal_value=1  Q_specify=off  Q_priority=None  Q=0 W  Q_nominal_specify=off  Q_nominal_unit=W  Q_nominal_value=1
      settings: SourceProductName=Simscape  SourceProductBaseCode=SS
  R_toER(2.1) : fl_lib/Thermal/Thermal Elements/Thermal Resistance  resistance=R_toER K/W  T_specify=off  T_priority=None  T=0 K  T_nominal_specify=off  T_nominal_unit=K  T_nominal_value=1  Q_specify=off  Q_priority=None  Q=0 W  Q_nominal_specify=off  Q_nominal_unit=W  Q_nominal_value=1
      settings: SourceProductName=Simscape  SourceProductBaseCode=SS
  R_toER(2.2) : fl_lib/Thermal/Thermal Elements/Thermal Resistance  resistance=R_toER K/W  T_specify=off  T_priority=None  T=0 K  T_nominal_specify=off  T_nominal_unit=K  T_nominal_value=1  Q_specify=off  Q_priority=None  Q=0 W  Q_nominal_specify=off  Q_nominal_unit=W  Q_nominal_value=1
      settings: SourceProductName=Simscape  SourceProductBaseCode=SS
  R_toER(3.1) : fl_lib/Thermal/Thermal Elements/Thermal Resistance  resistance=R_toER K/W  T_specify=off  T_priority=None  T=0 K  T_nominal_specify=off  T_nominal_unit=K  T_nominal_value=1  Q_specify=off  Q_priority=None  Q=0 W  Q_nominal_specify=off  Q_nominal_unit=W  Q_nominal_value=1
      settings: SourceProductName=Simscape  SourceProductBaseCode=SS
  R_toER(3.2) : fl_lib/Thermal/Thermal Elements/Thermal Resistance  resistance=R_toER K/W  T_specify=off  T_priority=None  T=0 K  T_nominal_specify=off  T_nominal_unit=K  T_nominal_value=1  Q_specify=off  Q_priority=None  Q=0 W  Q_nominal_specify=off  Q_nominal_unit=W  Q_nominal_value=1
      settings: SourceProductName=Simscape  SourceProductBaseCode=SS
  R_toER(4.1) : fl_lib/Thermal/Thermal Elements/Thermal Resistance  resistance=R_toER K/W  T_specify=off  T_priority=None  T=0 K  T_nominal_specify=off  T_nominal_unit=K  T_nominal_value=1  Q_specify=off  Q_priority=None  Q=0 W  Q_nominal_specify=off  Q_nominal_unit=W  Q_nominal_value=1
      settings: SourceProductName=Simscape  SourceProductBaseCode=SS
  R_toER(4.2) : fl_lib/Thermal/Thermal Elements/Thermal Resistance  resistance=R_toER K/W  T_specify=off  T_priority=None  T=0 K  T_nominal_specify=off  T_nominal_unit=K  T_nominal_value=1  Q_specify=off  Q_priority=None  Q=0 W  Q_nominal_specify=off  Q_nominal_unit=W  Q_nominal_value=1
      settings: SourceProductName=Simscape  SourceProductBaseCode=SS
  R_toER(5.1) : fl_lib/Thermal/Thermal Elements/Thermal Resistance  resistance=R_toER K/W  T_specify=off  T_priority=None  T=0 K  T_nominal_specify=off  T_nominal_unit=K  T_nominal_value=1  Q_specify=off  Q_priority=None  Q=0 W  Q_nominal_specify=off  Q_nominal_unit=W  Q_nominal_value=1
      settings: SourceProductName=Simscape  SourceProductBaseCode=SS
  R_toER(5.2) : fl_lib/Thermal/Thermal Elements/Thermal Resistance  resistance=R_toER K/W  T_specify=off  T_priority=None  T=0 K  T_nominal_specify=off  T_nominal_unit=K  T_nominal_value=1  Q_specify=off  Q_priority=None  Q=0 W  Q_nominal_specify=off  Q_nominal_unit=W  Q_nominal_value=1
      settings: SourceProductName=Simscape  SourceProductBaseCode=SS
  R_toHO(1) : fl_lib/Thermal/Thermal Elements/Thermal Resistance  resistance=R_toHO K/W  T_specify=off  T_priority=None  T=0 K  T_nominal_specify=off  T_nominal_unit=K  T_nominal_value=1  Q_specify=off  Q_priority=None  Q=0 W  Q_nominal_specify=off  Q_nominal_unit=W  Q_nominal_value=1
      settings: SourceProductName=Simscape  SourceProductBaseCode=SS
  R_toHO(2) : fl_lib/Thermal/Thermal Elements/Thermal Resistance  resistance=R_toHO K/W  T_specify=off  T_priority=None  T=0 K  T_nominal_specify=off  T_nominal_unit=K  T_nominal_value=1  Q_specify=off  Q_priority=None  Q=0 W  Q_nominal_specify=off  Q_nominal_unit=W  Q_nominal_value=1
      settings: SourceProductName=Simscape  SourceProductBaseCode=SS
  R_toHO(3) : fl_lib/Thermal/Thermal Elements/Thermal Resistance  resistance=R_toHO K/W  T_specify=off  T_priority=None  T=0 K  T_nominal_specify=off  T_nominal_unit=K  T_nominal_value=1  Q_specify=off  Q_priority=None  Q=0 W  Q_nominal_specify=off  Q_nominal_unit=W  Q_nominal_value=1
      settings: SourceProductName=Simscape  SourceProductBaseCode=SS
  R_toHO(4) : fl_lib/Thermal/Thermal Elements/Thermal Resistance  resistance=R_toHO K/W  T_specify=off  T_priority=None  T=0 K  T_nominal_specify=off  T_nominal_unit=K  T_nominal_value=1  Q_specify=off  Q_priority=None  Q=0 W  Q_nominal_specify=off  Q_nominal_unit=W  Q_nominal_value=1
      settings: SourceProductName=Simscape  SourceProductBaseCode=SS
  R_toHO(5) : fl_lib/Thermal/Thermal Elements/Thermal Resistance  resistance=R_toHO K/W  T_specify=off  T_priority=None  T=0 K  T_nominal_specify=off  T_nominal_unit=K  T_nominal_value=1  Q_specify=off  Q_priority=None  Q=0 W  Q_nominal_specify=off  Q_nominal_unit=W  Q_nominal_value=1
      settings: SourceProductName=Simscape  SourceProductBaseCode=SS
  R_toHO2(1) : fl_lib/Thermal/Thermal Elements/Thermal Resistance  resistance=R_toHO2 K/W  T_specify=off  T_priority=None  T=0 K  T_nominal_specify=off  T_nominal_unit=K  T_nominal_value=1  Q_specify=off  Q_priority=None  Q=0 W  Q_nominal_specify=off  Q_nominal_unit=W  Q_nominal_value=1
      settings: SourceProductName=Simscape  SourceProductBaseCode=SS
  R_toHO2(2) : fl_lib/Thermal/Thermal Elements/Thermal Resistance  resistance=R_toHO2 K/W  T_specify=off  T_priority=None  T=0 K  T_nominal_specify=off  T_nominal_unit=K  T_nominal_value=1  Q_specify=off  Q_priority=None  Q=0 W  Q_nominal_specify=off  Q_nominal_unit=W  Q_nominal_value=1
      settings: SourceProductName=Simscape  SourceProductBaseCode=SS
  R_toIA(1) : fl_lib/Thermal/Thermal Elements/Thermal Resistance  resistance=R_toIA K/W  T_specify=off  T_priority=None  T=0 K  T_nominal_specify=off  T_nominal_unit=K  T_nominal_value=1  Q_specify=off  Q_priority=None  Q=0 W  Q_nominal_specify=off  Q_nominal_unit=W  Q_nominal_value=1
      settings: SourceProductName=Simscape  SourceProductBaseCode=SS
  R_toIA(2) : fl_lib/Thermal/Thermal Elements/Thermal Resistance  resistance=R_toIA K/W  T_specify=off  T_priority=None  T=0 K  T_nominal_specify=off  T_nominal_unit=K  T_nominal_value=1  Q_specify=off  Q_priority=None  Q=0 W  Q_nominal_specify=off  Q_nominal_unit=W  Q_nominal_value=1
      settings: SourceProductName=Simscape  SourceProductBaseCode=SS
  R_toIA2(1) : fl_lib/Thermal/Thermal Elements/Thermal Resistance  resistance=R_toIA2 K/W  T_specify=off  T_priority=None  T=0 K  T_nominal_specify=off  T_nominal_unit=K  T_nominal_value=1  Q_specify=off  Q_priority=None  Q=0 W  Q_nominal_specify=off  Q_nominal_unit=W  Q_nominal_value=1
      settings: SourceProductName=Simscape  SourceProductBaseCode=SS
  R_toIA2(2) : fl_lib/Thermal/Thermal Elements/Thermal Resistance  resistance=R_toIA2 K/W  T_specify=off  T_priority=None  T=0 K  T_nominal_specify=off  T_nominal_unit=K  T_nominal_value=1  Q_specify=off  Q_priority=None  Q=0 W  Q_nominal_specify=off  Q_nominal_unit=W  Q_nominal_value=1
      settings: SourceProductName=Simscape  SourceProductBaseCode=SS
  R_toIA3(1) : fl_lib/Thermal/Thermal Elements/Thermal Resistance  resistance=R_toIA3 K/W  T_specify=off  T_priority=None  T=0 K  T_nominal_specify=off  T_nominal_unit=K  T_nominal_value=1  Q_specify=off  Q_priority=None  Q=0 W  Q_nominal_specify=off  Q_nominal_unit=W  Q_nominal_value=1
      settings: SourceProductName=Simscape  SourceProductBaseCode=SS
  R_toIA3(2) : fl_lib/Thermal/Thermal Elements/Thermal Resistance  resistance=R_toIA3 K/W  T_specify=off  T_priority=None  T=0 K  T_nominal_specify=off  T_nominal_unit=K  T_nominal_value=1  Q_specify=off  Q_priority=None  Q=0 W  Q_nominal_specify=off  Q_nominal_unit=W  Q_nominal_value=1
      settings: SourceProductName=Simscape  SourceProductBaseCode=SS
  R_toIA4(1)1 : fl_lib/Thermal/Thermal Elements/Thermal Resistance  resistance=R_toIA4 K/W  T_specify=off  T_priority=None  T=0 K  T_nominal_specify=off  T_nominal_unit=K  T_nominal_value=1  Q_specify=off  Q_priority=None  Q=0 W  Q_nominal_specify=off  Q_nominal_unit=W  Q_nominal_value=1
      settings: SourceProductName=Simscape  SourceProductBaseCode=SS
  R_toIA4(2) : fl_lib/Thermal/Thermal Elements/Thermal Resistance  resistance=R_toIA4 K/W  T_specify=off  T_priority=None  T=0 K  T_nominal_specify=off  T_nominal_unit=K  T_nominal_value=1  Q_specify=off  Q_priority=None  Q=0 W  Q_nominal_specify=off  Q_nominal_unit=W  Q_nominal_value=1
      settings: SourceProductName=Simscape  SourceProductBaseCode=SS
  R_toIA5(1) : fl_lib/Thermal/Thermal Elements/Thermal Resistance  resistance=R_toIA5 K/W  T_specify=off  T_priority=None  T=0 K  T_nominal_specify=off  T_nominal_unit=K  T_nominal_value=1  Q_specify=off  Q_priority=None  Q=0 W  Q_nominal_specify=off  Q_nominal_unit=W  Q_nominal_value=1
      settings: SourceProductName=Simscape  SourceProductBaseCode=SS
  R_toIA5(2) : fl_lib/Thermal/Thermal Elements/Thermal Resistance  resistance=R_toIA5 K/W  T_specify=off  T_priority=None  T=0 K  T_nominal_specify=off  T_nominal_unit=K  T_nominal_value=1  Q_specify=off  Q_priority=None  Q=0 W  Q_nominal_specify=off  Q_nominal_unit=W  Q_nominal_value=1
      settings: SourceProductName=Simscape  SourceProductBaseCode=SS
  R_toIA6(1) : fl_lib/Thermal/Thermal Elements/Thermal Resistance  resistance=R_toIA6 K/W  T_specify=off  T_priority=None  T=0 K  T_nominal_specify=off  T_nominal_unit=K  T_nominal_value=1  Q_specify=off  Q_priority=None  Q=0 W  Q_nominal_specify=off  Q_nominal_unit=W  Q_nominal_value=1
      settings: SourceProductName=Simscape  SourceProductBaseCode=SS
  R_toIA6(2) : fl_lib/Thermal/Thermal Elements/Thermal Resistance  resistance=R_toIA6 K/W  T_specify=off  T_priority=None  T=0 K  T_nominal_specify=off  T_nominal_unit=K  T_nominal_value=1  Q_specify=off  Q_priority=None  Q=0 W  Q_nominal_specify=off  Q_nominal_unit=W  Q_nominal_value=1
      settings: SourceProductName=Simscape  SourceProductBaseCode=SS
  R_toIA7(1) : fl_lib/Thermal/Thermal Elements/Thermal Resistance  resistance=R_toIA7 K/W  T_specify=off  T_priority=None  T=0 K  T_nominal_specify=off  T_nominal_unit=K  T_nominal_value=1  Q_specify=off  Q_priority=None  Q=0 W  Q_nominal_specify=off  Q_nominal_unit=W  Q_nominal_value=1
      settings: SourceProductName=Simscape  SourceProductBaseCode=SS
  R_toIA7(2) : fl_lib/Thermal/Thermal Elements/Thermal Resistance  resistance=R_toIA7 K/W  T_specify=off  T_priority=None  T=0 K  T_nominal_specify=off  T_nominal_unit=K  T_nominal_value=1  Q_specify=off  Q_priority=None  Q=0 W  Q_nominal_specify=off  Q_nominal_unit=W  Q_nominal_value=1
      settings: SourceProductName=Simscape  SourceProductBaseCode=SS
  R_toRAGP(1) : fl_lib/Thermal/Thermal Elements/Thermal Resistance  resistance=R_toRAGP K/W  T_specify=off  T_priority=None  T=0 K  T_nominal_specify=off  T_nominal_unit=K  T_nominal_value=1  Q_specify=off  Q_priority=None  Q=0 W  Q_nominal_specify=off  Q_nominal_unit=W  Q_nominal_value=1
      settings: SourceProductName=Simscape  SourceProductBaseCode=SS
  R_toRAGP(2) : fl_lib/Thermal/Thermal Elements/Thermal Resistance  resistance=R_toRAGP K/W  T_specify=off  T_priority=None  T=0 K  T_nominal_specify=off  T_nominal_unit=K  T_nominal_value=1  Q_specify=off  Q_priority=None  Q=0 W  Q_nominal_specify=off  Q_nominal_unit=W  Q_nominal_value=1
      settings: SourceProductName=Simscape  SourceProductBaseCode=SS
  R_toRAGP(3) : fl_lib/Thermal/Thermal Elements/Thermal Resistance  resistance=R_toRAGP K/W  T_specify=off  T_priority=None  T=0 K  T_nominal_specify=off  T_nominal_unit=K  T_nominal_value=1  Q_specify=off  Q_priority=None  Q=0 W  Q_nominal_specify=off  Q_nominal_unit=W  Q_nominal_value=1
      settings: SourceProductName=Simscape  SourceProductBaseCode=SS
  R_toRAGP(4) : fl_lib/Thermal/Thermal Elements/Thermal Resistance  resistance=R_toRAGP K/W  T_specify=off  T_priority=None  T=0 K  T_nominal_specify=off  T_nominal_unit=K  T_nominal_value=1  Q_specify=off  Q_priority=None  Q=0 W  Q_nominal_specify=off  Q_nominal_unit=W  Q_nominal_value=1
      settings: SourceProductName=Simscape  SourceProductBaseCode=SS
  R_toRAGP(5) : fl_lib/Thermal/Thermal Elements/Thermal Resistance  resistance=R_toRAGP K/W  T_specify=off  T_priority=None  T=0 K  T_nominal_specify=off  T_nominal_unit=K  T_nominal_value=1  Q_specify=off  Q_priority=None  Q=0 W  Q_nominal_specify=off  Q_nominal_unit=W  Q_nominal_value=1
      settings: SourceProductName=Simscape  SourceProductBaseCode=SS
  R_toRAGP2(1) : fl_lib/Thermal/Thermal Elements/Thermal Resistance  resistance=R_toRAGP2 K/W  T_specify=off  T_priority=None  T=0 K  T_nominal_specify=off  T_nominal_unit=K  T_nominal_value=1  Q_specify=off  Q_priority=None  Q=0 W  Q_nominal_specify=off  Q_nominal_unit=W  Q_nominal_value=1
      settings: SourceProductName=Simscape  SourceProductBaseCode=SS
  R_toRAGP2(2) : fl_lib/Thermal/Thermal Elements/Thermal Resistance  resistance=R_toRAGP2 K/W  T_specify=off  T_priority=None  T=0 K  T_nominal_specify=off  T_nominal_unit=K  T_nominal_value=1  Q_specify=off  Q_priority=None  Q=0 W  Q_nominal_specify=off  Q_nominal_unit=W  Q_nominal_value=1
      settings: SourceProductName=Simscape  SourceProductBaseCode=SS
  R_toRAGP2(3) : fl_lib/Thermal/Thermal Elements/Thermal Resistance  resistance=R_toRAGP2 K/W  T_specify=off  T_priority=None  T=0 K  T_nominal_specify=off  T_nominal_unit=K  T_nominal_value=1  Q_specify=off  Q_priority=None  Q=0 W  Q_nominal_specify=off  Q_nominal_unit=W  Q_nominal_value=1
      settings: SourceProductName=Simscape  SourceProductBaseCode=SS
  R_toRAGP2(4) : fl_lib/Thermal/Thermal Elements/Thermal Resistance  resistance=R_toRAGP2 K/W  T_specify=off  T_priority=None  T=0 K  T_nominal_specify=off  T_nominal_unit=K  T_nominal_value=1  Q_specify=off  Q_priority=None  Q=0 W  Q_nominal_specify=off  Q_nominal_unit=W  Q_nominal_value=1
      settings: SourceProductName=Simscape  SourceProductBaseCode=SS
  R_toRAGP2(5) : fl_lib/Thermal/Thermal Elements/Thermal Resistance  resistance=R_toRAGP2 K/W  T_specify=off  T_priority=None  T=0 K  T_nominal_specify=off  T_nominal_unit=K  T_nominal_value=1  Q_specify=off  Q_priority=None  Q=0 W  Q_nominal_specify=off  Q_nominal_unit=W  Q_nominal_value=1
      settings: SourceProductName=Simscape  SourceProductBaseCode=SS
  R_toRSL(1.1) : fl_lib/Thermal/Thermal Elements/Thermal Resistance  resistance=R_toRSL K/W  T_specify=off  T_priority=None  T=0 K  T_nominal_specify=off  T_nominal_unit=K  T_nominal_value=1  Q_specify=off  Q_priority=None  Q=0 W  Q_nominal_specify=off  Q_nominal_unit=W  Q_nominal_value=1
      settings: SourceProductName=Simscape  SourceProductBaseCode=SS
  R_toRSL(1.2) : fl_lib/Thermal/Thermal Elements/Thermal Resistance  resistance=R_toRSL K/W  T_specify=off  T_priority=None  T=0 K  T_nominal_specify=off  T_nominal_unit=K  T_nominal_value=1  Q_specify=off  Q_priority=None  Q=0 W  Q_nominal_specify=off  Q_nominal_unit=W  Q_nominal_value=1
      settings: SourceProductName=Simscape  SourceProductBaseCode=SS
  R_toRSL(2.1) : fl_lib/Thermal/Thermal Elements/Thermal Resistance  resistance=R_toRSL K/W  T_specify=off  T_priority=None  T=0 K  T_nominal_specify=off  T_nominal_unit=K  T_nominal_value=1  Q_specify=off  Q_priority=None  Q=0 W  Q_nominal_specify=off  Q_nominal_unit=W  Q_nominal_value=1
      settings: SourceProductName=Simscape  SourceProductBaseCode=SS
  R_toRSL(2.2) : fl_lib/Thermal/Thermal Elements/Thermal Resistance  resistance=R_toRSL K/W  T_specify=off  T_priority=None  T=0 K  T_nominal_specify=off  T_nominal_unit=K  T_nominal_value=1  Q_specify=off  Q_priority=None  Q=0 W  Q_nominal_specify=off  Q_nominal_unit=W  Q_nominal_value=1
      settings: SourceProductName=Simscape  SourceProductBaseCode=SS
  R_toRSL2(1) : fl_lib/Thermal/Thermal Elements/Thermal Resistance  resistance=R_toRSL2 K/W  T_specify=off  T_priority=None  T=0 K  T_nominal_specify=off  T_nominal_unit=K  T_nominal_value=1  Q_specify=off  Q_priority=None  Q=0 W  Q_nominal_specify=off  Q_nominal_unit=W  Q_nominal_value=1
      settings: SourceProductName=Simscape  SourceProductBaseCode=SS
  R_toRSL2(2) : fl_lib/Thermal/Thermal Elements/Thermal Resistance  resistance=R_toRSL2 K/W  T_specify=off  T_priority=None  T=0 K  T_nominal_specify=off  T_nominal_unit=K  T_nominal_value=1  Q_specify=off  Q_priority=None  Q=0 W  Q_nominal_specify=off  Q_nominal_unit=W  Q_nominal_value=1
      settings: SourceProductName=Simscape  SourceProductBaseCode=SS
  R_toRSL2(3) : fl_lib/Thermal/Thermal Elements/Thermal Resistance  resistance=R_toRSL2 K/W  T_specify=off  T_priority=None  T=0 K  T_nominal_specify=off  T_nominal_unit=K  T_nominal_value=1  Q_specify=off  Q_priority=None  Q=0 W  Q_nominal_specify=off  Q_nominal_unit=W  Q_nominal_value=1
      settings: SourceProductName=Simscape  SourceProductBaseCode=SS
  R_toRSL2(4) : fl_lib/Thermal/Thermal Elements/Thermal Resistance  resistance=R_toRSL2 K/W  T_specify=off  T_priority=None  T=0 K  T_nominal_specify=off  T_nominal_unit=K  T_nominal_value=1  Q_specify=off  Q_priority=None  Q=0 W  Q_nominal_specify=off  Q_nominal_unit=W  Q_nominal_value=1
      settings: SourceProductName=Simscape  SourceProductBaseCode=SS
  R_toRSL2(5) : fl_lib/Thermal/Thermal Elements/Thermal Resistance  resistance=R_toRSL2 K/W  T_specify=off  T_priority=None  T=0 K  T_nominal_specify=off  T_nominal_unit=K  T_nominal_value=1  Q_specify=off  Q_priority=None  Q=0 W  Q_nominal_specify=off  Q_nominal_unit=W  Q_nominal_value=1
      settings: SourceProductName=Simscape  SourceProductBaseCode=SS
  R_toRSLTO(1) : fl_lib/Thermal/Thermal Elements/Thermal Resistance  resistance=R_toRSLTO K/W  T_specify=off  T_priority=None  T=0 K  T_nominal_specify=off  T_nominal_unit=K  T_nominal_value=1  Q_specify=off  Q_priority=None  Q=0 W  Q_nominal_specify=off  Q_nominal_unit=W  Q_nominal_value=1
      settings: SourceProductName=Simscape  SourceProductBaseCode=SS
  R_toRSLTO(2) : fl_lib/Thermal/Thermal Elements/Thermal Resistance  resistance=R_toRSLTO K/W  T_specify=off  T_priority=None  T=0 K  T_nominal_specify=off  T_nominal_unit=K  T_nominal_value=1  Q_specify=off  Q_priority=None  Q=0 W  Q_nominal_specify=off  Q_nominal_unit=W  Q_nominal_value=1
      settings: SourceProductName=Simscape  SourceProductBaseCode=SS
  R_toRSLTO(3) : fl_lib/Thermal/Thermal Elements/Thermal Resistance  resistance=R_toRSLTO K/W  T_specify=off  T_priority=None  T=0 K  T_nominal_specify=off  T_nominal_unit=K  T_nominal_value=1  Q_specify=off  Q_priority=None  Q=0 W  Q_nominal_specify=off  Q_nominal_unit=W  Q_nominal_value=1
      settings: SourceProductName=Simscape  SourceProductBaseCode=SS
  R_toRSLTO(4) : fl_lib/Thermal/Thermal Elements/Thermal Resistance  resistance=R_toRSLTO K/W  T_specify=off  T_priority=None  T=0 K  T_nominal_specify=off  T_nominal_unit=K  T_nominal_value=1  Q_specify=off  Q_priority=None  Q=0 W  Q_nominal_specify=off  Q_nominal_unit=W  Q_nominal_value=1
      settings: SourceProductName=Simscape  SourceProductBaseCode=SS
  R_toRSLTO(5) : fl_lib/Thermal/Thermal Elements/Thermal Resistance  resistance=R_toRSLTO K/W  T_specify=off  T_priority=None  T=0 K  T_nominal_specify=off  T_nominal_unit=K  T_nominal_value=1  Q_specify=off  Q_priority=None  Q=0 W  Q_nominal_specify=off  Q_nominal_unit=W  Q_nominal_value=1
      settings: SourceProductName=Simscape  SourceProductBaseCode=SS
  R_toRTO(1) : fl_lib/Thermal/Thermal Elements/Thermal Resistance  resistance=R_toRTO K/W  T_specify=off  T_priority=None  T=0 K  T_nominal_specify=off  T_nominal_unit=K  T_nominal_value=1  Q_specify=off  Q_priority=None  Q=0 W  Q_nominal_specify=off  Q_nominal_unit=W  Q_nominal_value=1
      settings: SourceProductName=Simscape  SourceProductBaseCode=SS
  R_toRTO(2) : fl_lib/Thermal/Thermal Elements/Thermal Resistance  resistance=R_toRTO K/W  T_specify=off  T_priority=None  T=0 K  T_nominal_specify=off  T_nominal_unit=K  T_nominal_value=1  Q_specify=off  Q_priority=None  Q=0 W  Q_nominal_specify=off  Q_nominal_unit=W  Q_nominal_value=1
      settings: SourceProductName=Simscape  SourceProductBaseCode=SS
  R_toRTO(3) : fl_lib/Thermal/Thermal Elements/Thermal Resistance  resistance=R_toRTO K/W  T_specify=off  T_priority=None  T=0 K  T_nominal_specify=off  T_nominal_unit=K  T_nominal_value=1  Q_specify=off  Q_priority=None  Q=0 W  Q_nominal_specify=off  Q_nominal_unit=W  Q_nominal_value=1
      settings: SourceProductName=Simscape  SourceProductBaseCode=SS
  R_toRTO(4) : fl_lib/Thermal/Thermal Elements/Thermal Resistance  resistance=R_toRTO K/W  T_specify=off  T_priority=None  T=0 K  T_nominal_specify=off  T_nominal_unit=K  T_nominal_value=1  Q_specify=off  Q_priority=None  Q=0 W  Q_nominal_specify=off  Q_nominal_unit=W  Q_nominal_value=1
      settings: SourceProductName=Simscape  SourceProductBaseCode=SS
  R_toRTO(5) : fl_lib/Thermal/Thermal Elements/Thermal Resistance  resistance=R_toRTO K/W  T_specify=off  T_priority=None  T=0 K  T_nominal_specify=off  T_nominal_unit=K  T_nominal_value=1  Q_specify=off  Q_priority=None  Q=0 W  Q_nominal_specify=off  Q_nominal_unit=W  Q_nominal_value=1
      settings: SourceProductName=Simscape  SourceProductBaseCode=SS
  R_toRYO(1) : fl_lib/Thermal/Thermal Elements/Thermal Resistance  resistance=R_toRYO K/W  T_specify=off  T_priority=None  T=0 K  T_nominal_specify=off  T_nominal_unit=K  T_nominal_value=1  Q_specify=off  Q_priority=None  Q=0 W  Q_nominal_specify=off  Q_nominal_unit=W  Q_nominal_value=1
      settings: SourceProductName=Simscape  SourceProductBaseCode=SS
  R_toRYO(2) : fl_lib/Thermal/Thermal Elements/Thermal Resistance  resistance=R_toRYO K/W  T_specify=off  T_priority=None  T=0 K  T_nominal_specify=off  T_nominal_unit=K  T_nominal_value=1  Q_specify=off  Q_priority=None  Q=0 W  Q_nominal_specify=off  Q_nominal_unit=W  Q_nominal_value=1
      settings: SourceProductName=Simscape  SourceProductBaseCode=SS
  R_toRYO(3) : fl_lib/Thermal/Thermal Elements/Thermal Resistance  resistance=R_toRYO K/W  T_specify=off  T_priority=None  T=0 K  T_nominal_specify=off  T_nominal_unit=K  T_nominal_value=1  Q_specify=off  Q_priority=None  Q=0 W  Q_nominal_specify=off  Q_nominal_unit=W  Q_nominal_value=1
      settings: SourceProductName=Simscape  SourceProductBaseCode=SS
  R_toRYO(4) : fl_lib/Thermal/Thermal Elements/Thermal Resistance  resistance=R_toRYO K/W  T_specify=off  T_priority=None  T=0 K  T_nominal_specify=off  T_nominal_unit=K  T_nominal_value=1  Q_specify=off  Q_priority=None  Q=0 W  Q_nominal_specify=off  Q_nominal_unit=W  Q_nominal_value=1
      settings: SourceProductName=Simscape  SourceProductBaseCode=SS
  R_toRYO(5) : fl_lib/Thermal/Thermal Elements/Thermal Resistance  resistance=R_toRYO K/W  T_specify=off  T_priority=None  T=0 K  T_nominal_specify=off  T_nominal_unit=K  T_nominal_value=1  Q_specify=off  Q_priority=None  Q=0 W  Q_nominal_specify=off  Q_nominal_unit=W  Q_nominal_value=1
      settings: SourceProductName=Simscape  SourceProductBaseCode=SS
  R_toRYO2(1) : fl_lib/Thermal/Thermal Elements/Thermal Resistance  resistance=R_toRYO2 K/W  T_specify=off  T_priority=None  T=0 K  T_nominal_specify=off  T_nominal_unit=K  T_nominal_value=1  Q_specify=off  Q_priority=None  Q=0 W  Q_nominal_specify=off  Q_nominal_unit=W  Q_nominal_value=1
      settings: SourceProductName=Simscape  SourceProductBaseCode=SS
  R_toRYO2(2) : fl_lib/Thermal/Thermal Elements/Thermal Resistance  resistance=R_toRYO2 K/W  T_specify=off  T_priority=None  T=0 K  T_nominal_specify=off  T_nominal_unit=K  T_nominal_value=1  Q_specify=off  Q_priority=None  Q=0 W  Q_nominal_specify=off  Q_nominal_unit=W  Q_nominal_value=1
      settings: SourceProductName=Simscape  SourceProductBaseCode=SS
  R_toRYO2(3) : fl_lib/Thermal/Thermal Elements/Thermal Resistance  resistance=R_toRYO2 K/W  T_specify=off  T_priority=None  T=0 K  T_nominal_specify=off  T_nominal_unit=K  T_nominal_value=1  Q_specify=off  Q_priority=None  Q=0 W  Q_nominal_specify=off  Q_nominal_unit=W  Q_nominal_value=1
      settings: SourceProductName=Simscape  SourceProductBaseCode=SS
  R_toRYO2(4) : fl_lib/Thermal/Thermal Elements/Thermal Resistance  resistance=R_toRYO2 K/W  T_specify=off  T_priority=None  T=0 K  T_nominal_specify=off  T_nominal_unit=K  T_nominal_value=1  Q_specify=off  Q_priority=None  Q=0 W  Q_nominal_specify=off  Q_nominal_unit=W  Q_nominal_value=1
      settings: SourceProductName=Simscape  SourceProductBaseCode=SS
  R_toRYO2(5) : fl_lib/Thermal/Thermal Elements/Thermal Resistance  resistance=R_toRYO2 K/W  T_specify=off  T_priority=None  T=0 K  T_nominal_specify=off  T_nominal_unit=K  T_nominal_value=1  Q_specify=off  Q_priority=None  Q=0 W  Q_nominal_specify=off  Q_nominal_unit=W  Q_nominal_value=1
      settings: SourceProductName=Simscape  SourceProductBaseCode=SS
  R_toRYO3(1) : fl_lib/Thermal/Thermal Elements/Thermal Resistance  resistance=R_toRYO3 K/W  T_specify=off  T_priority=None  T=0 K  T_nominal_specify=off  T_nominal_unit=K  T_nominal_value=1  Q_specify=off  Q_priority=None  Q=0 W  Q_nominal_specify=off  Q_nominal_unit=W  Q_nominal_value=1
      settings: SourceProductName=Simscape  SourceProductBaseCode=SS
  R_toRYO3(2) : fl_lib/Thermal/Thermal Elements/Thermal Resistance  resistance=R_toRYO3 K/W  T_specify=off  T_priority=None  T=0 K  T_nominal_specify=off  T_nominal_unit=K  T_nominal_value=1  Q_specify=off  Q_priority=None  Q=0 W  Q_nominal_specify=off  Q_nominal_unit=W  Q_nominal_value=1
      settings: SourceProductName=Simscape  SourceProductBaseCode=SS
  R_toRYO3(3) : fl_lib/Thermal/Thermal Elements/Thermal Resistance  resistance=R_toRYO3 K/W  T_specify=off  T_priority=None  T=0 K  T_nominal_specify=off  T_nominal_unit=K  T_nominal_value=1  Q_specify=off  Q_priority=None  Q=0 W  Q_nominal_specify=off  Q_nominal_unit=W  Q_nominal_value=1
      settings: SourceProductName=Simscape  SourceProductBaseCode=SS
  R_toRYO3(4) : fl_lib/Thermal/Thermal Elements/Thermal Resistance  resistance=R_toRYO3 K/W  T_specify=off  T_priority=None  T=0 K  T_nominal_specify=off  T_nominal_unit=K  T_nominal_value=1  Q_specify=off  Q_priority=None  Q=0 W  Q_nominal_specify=off  Q_nominal_unit=W  Q_nominal_value=1
      settings: SourceProductName=Simscape  SourceProductBaseCode=SS
  R_toRYO3(5) : fl_lib/Thermal/Thermal Elements/Thermal Resistance  resistance=R_toRYO3 K/W  T_specify=off  T_priority=None  T=0 K  T_nominal_specify=off  T_nominal_unit=K  T_nominal_value=1  Q_specify=off  Q_priority=None  Q=0 W  Q_nominal_specify=off  Q_nominal_unit=W  Q_nominal_value=1
      settings: SourceProductName=Simscape  SourceProductBaseCode=SS
  R_toSAGP(1) : fl_lib/Thermal/Thermal Elements/Thermal Resistance  resistance=R_toSAGP K/W  T_specify=off  T_priority=None  T=0 K  T_nominal_specify=off  T_nominal_unit=K  T_nominal_value=1  Q_specify=off  Q_priority=None  Q=0 W  Q_nominal_specify=off  Q_nominal_unit=W  Q_nominal_value=1
      settings: SourceProductName=Simscape  SourceProductBaseCode=SS
  R_toSAGP(2) : fl_lib/Thermal/Thermal Elements/Thermal Resistance  resistance=R_toSAGP K/W  T_specify=off  T_priority=None  T=0 K  T_nominal_specify=off  T_nominal_unit=K  T_nominal_value=1  Q_specify=off  Q_priority=None  Q=0 W  Q_nominal_specify=off  Q_nominal_unit=W  Q_nominal_value=1
      settings: SourceProductName=Simscape  SourceProductBaseCode=SS
  R_toSAGP(3) : fl_lib/Thermal/Thermal Elements/Thermal Resistance  resistance=R_toSAGP K/W  T_specify=off  T_priority=None  T=0 K  T_nominal_specify=off  T_nominal_unit=K  T_nominal_value=1  Q_specify=off  Q_priority=None  Q=0 W  Q_nominal_specify=off  Q_nominal_unit=W  Q_nominal_value=1
      settings: SourceProductName=Simscape  SourceProductBaseCode=SS
  R_toSAGP(4) : fl_lib/Thermal/Thermal Elements/Thermal Resistance  resistance=R_toSAGP K/W  T_specify=off  T_priority=None  T=0 K  T_nominal_specify=off  T_nominal_unit=K  T_nominal_value=1  Q_specify=off  Q_priority=None  Q=0 W  Q_nominal_specify=off  Q_nominal_unit=W  Q_nominal_value=1
      settings: SourceProductName=Simscape  SourceProductBaseCode=SS
  R_toSAGP(5) : fl_lib/Thermal/Thermal Elements/Thermal Resistance  resistance=R_toSAGP K/W  T_specify=off  T_priority=None  T=0 K  T_nominal_specify=off  T_nominal_unit=K  T_nominal_value=1  Q_specify=off  Q_priority=None  Q=0 W  Q_nominal_specify=off  Q_nominal_unit=W  Q_nominal_value=1
      settings: SourceProductName=Simscape  SourceProductBaseCode=SS
  R_toSAGP2(1) : fl_lib/Thermal/Thermal Elements/Thermal Resistance  resistance=R_toSAGP2 K/W  T_specify=off  T_priority=None  T=0 K  T_nominal_specify=off  T_nominal_unit=K  T_nominal_value=1  Q_specify=off  Q_priority=None  Q=0 W  Q_nominal_specify=off  Q_nominal_unit=W  Q_nominal_value=1
      settings: SourceProductName=Simscape  SourceProductBaseCode=SS
  R_toSAGP2(2) : fl_lib/Thermal/Thermal Elements/Thermal Resistance  resistance=R_toSAGP2 K/W  T_specify=off  T_priority=None  T=0 K  T_nominal_specify=off  T_nominal_unit=K  T_nominal_value=1  Q_specify=off  Q_priority=None  Q=0 W  Q_nominal_specify=off  Q_nominal_unit=W  Q_nominal_value=1
      settings: SourceProductName=Simscape  SourceProductBaseCode=SS
  R_toSAGP2(3) : fl_lib/Thermal/Thermal Elements/Thermal Resistance  resistance=R_toSAGP2 K/W  T_specify=off  T_priority=None  T=0 K  T_nominal_specify=off  T_nominal_unit=K  T_nominal_value=1  Q_specify=off  Q_priority=None  Q=0 W  Q_nominal_specify=off  Q_nominal_unit=W  Q_nominal_value=1
      settings: SourceProductName=Simscape  SourceProductBaseCode=SS
  R_toSAGP2(4) : fl_lib/Thermal/Thermal Elements/Thermal Resistance  resistance=R_toSAGP2 K/W  T_specify=off  T_priority=None  T=0 K  T_nominal_specify=off  T_nominal_unit=K  T_nominal_value=1  Q_specify=off  Q_priority=None  Q=0 W  Q_nominal_specify=off  Q_nominal_unit=W  Q_nominal_value=1
      settings: SourceProductName=Simscape  SourceProductBaseCode=SS
  R_toSAGP2(5) : fl_lib/Thermal/Thermal Elements/Thermal Resistance  resistance=R_toSAGP2 K/W  T_specify=off  T_priority=None  T=0 K  T_nominal_specify=off  T_nominal_unit=K  T_nominal_value=1  Q_specify=off  Q_priority=None  Q=0 W  Q_nominal_specify=off  Q_nominal_unit=W  Q_nominal_value=1
      settings: SourceProductName=Simscape  SourceProductBaseCode=SS
  R_toSH(1) : fl_lib/Thermal/Thermal Elements/Thermal Resistance  resistance=R_toSH K/W  T_specify=off  T_priority=None  T=0 K  T_nominal_specify=off  T_nominal_unit=K  T_nominal_value=1  Q_specify=off  Q_priority=None  Q=0 W  Q_nominal_specify=off  Q_nominal_unit=W  Q_nominal_value=1
      settings: SourceProductName=Simscape  SourceProductBaseCode=SS
  R_toSH(2) : fl_lib/Thermal/Thermal Elements/Thermal Resistance  resistance=R_toSH K/W  T_specify=off  T_priority=None  T=0 K  T_nominal_specify=off  T_nominal_unit=K  T_nominal_value=1  Q_specify=off  Q_priority=None  Q=0 W  Q_nominal_specify=off  Q_nominal_unit=W  Q_nominal_value=1
      settings: SourceProductName=Simscape  SourceProductBaseCode=SS
  R_toSH(3) : fl_lib/Thermal/Thermal Elements/Thermal Resistance  resistance=R_toSH K/W  T_specify=off  T_priority=None  T=0 K  T_nominal_specify=off  T_nominal_unit=K  T_nominal_value=1  Q_specify=off  Q_priority=None  Q=0 W  Q_nominal_specify=off  Q_nominal_unit=W  Q_nominal_value=1
      settings: SourceProductName=Simscape  SourceProductBaseCode=SS
  R_toSH(4) : fl_lib/Thermal/Thermal Elements/Thermal Resistance  resistance=R_toSH K/W  T_specify=off  T_priority=None  T=0 K  T_nominal_specify=off  T_nominal_unit=K  T_nominal_value=1  Q_specify=off  Q_priority=None  Q=0 W  Q_nominal_specify=off  Q_nominal_unit=W  Q_nominal_value=1
      settings: SourceProductName=Simscape  SourceProductBaseCode=SS
  R_toSH(5) : fl_lib/Thermal/Thermal Elements/Thermal Resistance  resistance=R_toSH K/W  T_specify=off  T_priority=None  T=0 K  T_nominal_specify=off  T_nominal_unit=K  T_nominal_value=1  Q_specify=off  Q_priority=None  Q=0 W  Q_nominal_specify=off  Q_nominal_unit=W  Q_nominal_value=1
      settings: SourceProductName=Simscape  SourceProductBaseCode=SS
  R_toSSL(1.1) : fl_lib/Thermal/Thermal Elements/Thermal Resistance  resistance=R_toSSL K/W  T_specify=off  T_priority=None  T=0 K  T_nominal_specify=off  T_nominal_unit=K  T_nominal_value=1  Q_specify=off  Q_priority=None  Q=0 W  Q_nominal_specify=off  Q_nominal_unit=W  Q_nominal_value=1
      settings: SourceProductName=Simscape  SourceProductBaseCode=SS
  R_toSSL(1.2) : fl_lib/Thermal/Thermal Elements/Thermal Resistance  resistance=R_toSSL K/W  T_specify=off  T_priority=None  T=0 K  T_nominal_specify=off  T_nominal_unit=K  T_nominal_value=1  Q_specify=off  Q_priority=None  Q=0 W  Q_nominal_specify=off  Q_nominal_unit=W  Q_nominal_value=1
      settings: SourceProductName=Simscape  SourceProductBaseCode=SS
  R_toSSL(2.1) : fl_lib/Thermal/Thermal Elements/Thermal Resistance  resistance=R_toSSL K/W  T_specify=off  T_priority=None  T=0 K  T_nominal_specify=off  T_nominal_unit=K  T_nominal_value=1  Q_specify=off  Q_priority=None  Q=0 W  Q_nominal_specify=off  Q_nominal_unit=W  Q_nominal_value=1
      settings: SourceProductName=Simscape  SourceProductBaseCode=SS
  R_toSSL(2.2) : fl_lib/Thermal/Thermal Elements/Thermal Resistance  resistance=R_toSSL K/W  T_specify=off  T_priority=None  T=0 K  T_nominal_specify=off  T_nominal_unit=K  T_nominal_value=1  Q_specify=off  Q_priority=None  Q=0 W  Q_nominal_specify=off  Q_nominal_unit=W  Q_nominal_value=1
      settings: SourceProductName=Simscape  SourceProductBaseCode=SS
  R_toSSL2(1) : fl_lib/Thermal/Thermal Elements/Thermal Resistance  resistance=R_toSSL2 K/W  T_specify=off  T_priority=None  T=0 K  T_nominal_specify=off  T_nominal_unit=K  T_nominal_value=1  Q_specify=off  Q_priority=None  Q=0 W  Q_nominal_specify=off  Q_nominal_unit=W  Q_nominal_value=1
      settings: SourceProductName=Simscape  SourceProductBaseCode=SS
  R_toSSL2(2) : fl_lib/Thermal/Thermal Elements/Thermal Resistance  resistance=R_toSSL2 K/W  T_specify=off  T_priority=None  T=0 K  T_nominal_specify=off  T_nominal_unit=K  T_nominal_value=1  Q_specify=off  Q_priority=None  Q=0 W  Q_nominal_specify=off  Q_nominal_unit=W  Q_nominal_value=1
      settings: SourceProductName=Simscape  SourceProductBaseCode=SS
  R_toSSL2(3) : fl_lib/Thermal/Thermal Elements/Thermal Resistance  resistance=R_toSSL2 K/W  T_specify=off  T_priority=None  T=0 K  T_nominal_specify=off  T_nominal_unit=K  T_nominal_value=1  Q_specify=off  Q_priority=None  Q=0 W  Q_nominal_specify=off  Q_nominal_unit=W  Q_nominal_value=1
      settings: SourceProductName=Simscape  SourceProductBaseCode=SS
  R_toSSL2(4) : fl_lib/Thermal/Thermal Elements/Thermal Resistance  resistance=R_toSSL2 K/W  T_specify=off  T_priority=None  T=0 K  T_nominal_specify=off  T_nominal_unit=K  T_nominal_value=1  Q_specify=off  Q_priority=None  Q=0 W  Q_nominal_specify=off  Q_nominal_unit=W  Q_nominal_value=1
      settings: SourceProductName=Simscape  SourceProductBaseCode=SS
  R_toSSL2(5) : fl_lib/Thermal/Thermal Elements/Thermal Resistance  resistance=R_toSSL2 K/W  T_specify=off  T_priority=None  T=0 K  T_nominal_specify=off  T_nominal_unit=K  T_nominal_value=1  Q_specify=off  Q_priority=None  Q=0 W  Q_nominal_specify=off  Q_nominal_unit=W  Q_nominal_value=1
      settings: SourceProductName=Simscape  SourceProductBaseCode=SS
  R_toSSLTO(1) : fl_lib/Thermal/Thermal Elements/Thermal Resistance  resistance=R_toSSLTO K/W  T_specify=off  T_priority=None  T=0 K  T_nominal_specify=off  T_nominal_unit=K  T_nominal_value=1  Q_specify=off  Q_priority=None  Q=0 W  Q_nominal_specify=off  Q_nominal_unit=W  Q_nominal_value=1
      settings: SourceProductName=Simscape  SourceProductBaseCode=SS
  R_toSSLTO(2) : fl_lib/Thermal/Thermal Elements/Thermal Resistance  resistance=R_toSSLTO K/W  T_specify=off  T_priority=None  T=0 K  T_nominal_specify=off  T_nominal_unit=K  T_nominal_value=1  Q_specify=off  Q_priority=None  Q=0 W  Q_nominal_specify=off  Q_nominal_unit=W  Q_nominal_value=1
      settings: SourceProductName=Simscape  SourceProductBaseCode=SS
  R_toSSLTO(3) : fl_lib/Thermal/Thermal Elements/Thermal Resistance  resistance=R_toSSLTO K/W  T_specify=off  T_priority=None  T=0 K  T_nominal_specify=off  T_nominal_unit=K  T_nominal_value=1  Q_specify=off  Q_priority=None  Q=0 W  Q_nominal_specify=off  Q_nominal_unit=W  Q_nominal_value=1
      settings: SourceProductName=Simscape  SourceProductBaseCode=SS
  R_toSSLTO(4) : fl_lib/Thermal/Thermal Elements/Thermal Resistance  resistance=R_toSSLTO K/W  T_specify=off  T_priority=None  T=0 K  T_nominal_specify=off  T_nominal_unit=K  T_nominal_value=1  Q_specify=off  Q_priority=None  Q=0 W  Q_nominal_specify=off  Q_nominal_unit=W  Q_nominal_value=1
      settings: SourceProductName=Simscape  SourceProductBaseCode=SS
  R_toSSLTO(5) : fl_lib/Thermal/Thermal Elements/Thermal Resistance  resistance=R_toSSLTO K/W  T_specify=off  T_priority=None  T=0 K  T_nominal_specify=off  T_nominal_unit=K  T_nominal_value=1  Q_specify=off  Q_priority=None  Q=0 W  Q_nominal_specify=off  Q_nominal_unit=W  Q_nominal_value=1
      settings: SourceProductName=Simscape  SourceProductBaseCode=SS
  R_toSTO(1) : fl_lib/Thermal/Thermal Elements/Thermal Resistance  resistance=R_toSTO K/W  T_specify=off  T_priority=None  T=0 K  T_nominal_specify=off  T_nominal_unit=K  T_nominal_value=1  Q_specify=off  Q_priority=None  Q=0 W  Q_nominal_specify=off  Q_nominal_unit=W  Q_nominal_value=1
      settings: SourceProductName=Simscape  SourceProductBaseCode=SS
  R_toSTO(2) : fl_lib/Thermal/Thermal Elements/Thermal Resistance  resistance=R_toSTO K/W  T_specify=off  T_priority=None  T=0 K  T_nominal_specify=off  T_nominal_unit=K  T_nominal_value=1  Q_specify=off  Q_priority=None  Q=0 W  Q_nominal_specify=off  Q_nominal_unit=W  Q_nominal_value=1
      settings: SourceProductName=Simscape  SourceProductBaseCode=SS
  R_toSTO(3) : fl_lib/Thermal/Thermal Elements/Thermal Resistance  resistance=R_toSTO K/W  T_specify=off  T_priority=None  T=0 K  T_nominal_specify=off  T_nominal_unit=K  T_nominal_value=1  Q_specify=off  Q_priority=None  Q=0 W  Q_nominal_specify=off  Q_nominal_unit=W  Q_nominal_value=1
      settings: SourceProductName=Simscape  SourceProductBaseCode=SS
  R_toSTO(4) : fl_lib/Thermal/Thermal Elements/Thermal Resistance  resistance=R_toSTO K/W  T_specify=off  T_priority=None  T=0 K  T_nominal_specify=off  T_nominal_unit=K  T_nominal_value=1  Q_specify=off  Q_priority=None  Q=0 W  Q_nominal_specify=off  Q_nominal_unit=W  Q_nominal_value=1
      settings: SourceProductName=Simscape  SourceProductBaseCode=SS
  R_toSTO(5) : fl_lib/Thermal/Thermal Elements/Thermal Resistance  resistance=R_toSTO K/W  T_specify=off  T_priority=None  T=0 K  T_nominal_specify=off  T_nominal_unit=K  T_nominal_value=1  Q_specify=off  Q_priority=None  Q=0 W  Q_nominal_specify=off  Q_nominal_unit=W  Q_nominal_value=1
      settings: SourceProductName=Simscape  SourceProductBaseCode=SS
  R_toSYO(1) : fl_lib/Thermal/Thermal Elements/Thermal Resistance  resistance=R_toSYO K/W  T_specify=off  T_priority=None  T=0 K  T_nominal_specify=off  T_nominal_unit=K  T_nominal_value=1  Q_specify=off  Q_priority=None  Q=0 W  Q_nominal_specify=off  Q_nominal_unit=W  Q_nominal_value=1
      settings: SourceProductName=Simscape  SourceProductBaseCode=SS
  R_toSYO(2) : fl_lib/Thermal/Thermal Elements/Thermal Resistance  resistance=R_toSYO K/W  T_specify=off  T_priority=None  T=0 K  T_nominal_specify=off  T_nominal_unit=K  T_nominal_value=1  Q_specify=off  Q_priority=None  Q=0 W  Q_nominal_specify=off  Q_nominal_unit=W  Q_nominal_value=1
      settings: SourceProductName=Simscape  SourceProductBaseCode=SS
  R_toSYO(3) : fl_lib/Thermal/Thermal Elements/Thermal Resistance  resistance=R_toSYO K/W  T_specify=off  T_priority=None  T=0 K  T_nominal_specify=off  T_nominal_unit=K  T_nominal_value=1  Q_specify=off  Q_priority=None  Q=0 W  Q_nominal_specify=off  Q_nominal_unit=W  Q_nominal_value=1
      settings: SourceProductName=Simscape  SourceProductBaseCode=SS
  R_toSYO(4) : fl_lib/Thermal/Thermal Elements/Thermal Resistance  resistance=R_toSYO K/W  T_specify=off  T_priority=None  T=0 K  T_nominal_specify=off  T_nominal_unit=K  T_nominal_value=1  Q_specify=off  Q_priority=None  Q=0 W  Q_nominal_specify=off  Q_nominal_unit=W  Q_nominal_value=1
      settings: SourceProductName=Simscape  SourceProductBaseCode=SS
  R_toSYO(5) : fl_lib/Thermal/Thermal Elements/Thermal Resistance  resistance=R_toSYO K/W  T_specify=off  T_priority=None  T=0 K  T_nominal_specify=off  T_nominal_unit=K  T_nominal_value=1  Q_specify=off  Q_priority=None  Q=0 W  Q_nominal_specify=off  Q_nominal_unit=W  Q_nominal_value=1
      settings: SourceProductName=Simscape  SourceProductBaseCode=SS
  R_toSYO2(1) : fl_lib/Thermal/Thermal Elements/Thermal Resistance  resistance=R_toSYO2 K/W  T_specify=off  T_priority=None  T=0 K  T_nominal_specify=off  T_nominal_unit=K  T_nominal_value=1  Q_specify=off  Q_priority=None  Q=0 W  Q_nominal_specify=off  Q_nominal_unit=W  Q_nominal_value=1
      settings: SourceProductName=Simscape  SourceProductBaseCode=SS
  R_toSYO2(2) : fl_lib/Thermal/Thermal Elements/Thermal Resistance  resistance=R_toSYO2 K/W  T_specify=off  T_priority=None  T=0 K  T_nominal_specify=off  T_nominal_unit=K  T_nominal_value=1  Q_specify=off  Q_priority=None  Q=0 W  Q_nominal_specify=off  Q_nominal_unit=W  Q_nominal_value=1
      settings: SourceProductName=Simscape  SourceProductBaseCode=SS
  R_toSYO2(3) : fl_lib/Thermal/Thermal Elements/Thermal Resistance  resistance=R_toSYO2 K/W  T_specify=off  T_priority=None  T=0 K  T_nominal_specify=off  T_nominal_unit=K  T_nominal_value=1  Q_specify=off  Q_priority=None  Q=0 W  Q_nominal_specify=off  Q_nominal_unit=W  Q_nominal_value=1
      settings: SourceProductName=Simscape  SourceProductBaseCode=SS
  R_toSYO2(4) : fl_lib/Thermal/Thermal Elements/Thermal Resistance  resistance=R_toSYO2 K/W  T_specify=off  T_priority=None  T=0 K  T_nominal_specify=off  T_nominal_unit=K  T_nominal_value=1  Q_specify=off  Q_priority=None  Q=0 W  Q_nominal_specify=off  Q_nominal_unit=W  Q_nominal_value=1
      settings: SourceProductName=Simscape  SourceProductBaseCode=SS
  R_toSYO2(5) : fl_lib/Thermal/Thermal Elements/Thermal Resistance  resistance=R_toSYO2 K/W  T_specify=off  T_priority=None  T=0 K  T_nominal_specify=off  T_nominal_unit=K  T_nominal_value=1  Q_specify=off  Q_priority=None  Q=0 W  Q_nominal_specify=off  Q_nominal_unit=W  Q_nominal_value=1
      settings: SourceProductName=Simscape  SourceProductBaseCode=SS
  R_toSYO3(1) : fl_lib/Thermal/Thermal Elements/Thermal Resistance  resistance=R_toSYO3 K/W  T_specify=off  T_priority=None  T=0 K  T_nominal_specify=off  T_nominal_unit=K  T_nominal_value=1  Q_specify=off  Q_priority=None  Q=0 W  Q_nominal_specify=off  Q_nominal_unit=W  Q_nominal_value=1
      settings: SourceProductName=Simscape  SourceProductBaseCode=SS
  R_toSYO3(2) : fl_lib/Thermal/Thermal Elements/Thermal Resistance  resistance=R_toSYO3 K/W  T_specify=off  T_priority=None  T=0 K  T_nominal_specify=off  T_nominal_unit=K  T_nominal_value=1  Q_specify=off  Q_priority=None  Q=0 W  Q_nominal_specify=off  Q_nominal_unit=W  Q_nominal_value=1
      settings: SourceProductName=Simscape  SourceProductBaseCode=SS
  R_toSYO3(3) : fl_lib/Thermal/Thermal Elements/Thermal Resistance  resistance=R_toSYO3 K/W  T_specify=off  T_priority=None  T=0 K  T_nominal_specify=off  T_nominal_unit=K  T_nominal_value=1  Q_specify=off  Q_priority=None  Q=0 W  Q_nominal_specify=off  Q_nominal_unit=W  Q_nominal_value=1
      settings: SourceProductName=Simscape  SourceProductBaseCode=SS
  R_toSYO3(4) : fl_lib/Thermal/Thermal Elements/Thermal Resistance  resistance=R_toSYO3 K/W  T_specify=off  T_priority=None  T=0 K  T_nominal_specify=off  T_nominal_unit=K  T_nominal_value=1  Q_specify=off  Q_priority=None  Q=0 W  Q_nominal_specify=off  Q_nominal_unit=W  Q_nominal_value=1
      settings: SourceProductName=Simscape  SourceProductBaseCode=SS
  R_toSYO3(5) : fl_lib/Thermal/Thermal Elements/Thermal Resistance  resistance=R_toSYO3 K/W  T_specify=off  T_priority=None  T=0 K  T_nominal_specify=off  T_nominal_unit=K  T_nominal_value=1  Q_specify=off  Q_priority=None  Q=0 W  Q_nominal_specify=off  Q_nominal_unit=W  Q_nominal_value=1
      settings: SourceProductName=Simscape  SourceProductBaseCode=SS
  R_toWC_a(1) : fl_lib/Thermal/Thermal Elements/Thermal Resistance  resistance=R_toWC_a K/W  T_specify=off  T_priority=None  T=0 K  T_nominal_specify=off  T_nominal_unit=K  T_nominal_value=1  Q_specify=off  Q_priority=None  Q=0 W  Q_nominal_specify=off  Q_nominal_unit=W  Q_nominal_value=1
      settings: SourceProductName=Simscape  SourceProductBaseCode=SS
  R_toWC_a(2) : fl_lib/Thermal/Thermal Elements/Thermal Resistance  resistance=R_toWC_a K/W  T_specify=off  T_priority=None  T=0 K  T_nominal_specify=off  T_nominal_unit=K  T_nominal_value=1  Q_specify=off  Q_priority=None  Q=0 W  Q_nominal_specify=off  Q_nominal_unit=W  Q_nominal_value=1
      settings: SourceProductName=Simscape  SourceProductBaseCode=SS
  R_toWC_a(3) : fl_lib/Thermal/Thermal Elements/Thermal Resistance  resistance=R_toWC_a K/W  T_specify=off  T_priority=None  T=0 K  T_nominal_specify=off  T_nominal_unit=K  T_nominal_value=1  Q_specify=off  Q_priority=None  Q=0 W  Q_nominal_specify=off  Q_nominal_unit=W  Q_nominal_value=1
      settings: SourceProductName=Simscape  SourceProductBaseCode=SS
  R_toWC_a(4) : fl_lib/Thermal/Thermal Elements/Thermal Resistance  resistance=R_toWC_a K/W  T_specify=off  T_priority=None  T=0 K  T_nominal_specify=off  T_nominal_unit=K  T_nominal_value=1  Q_specify=off  Q_priority=None  Q=0 W  Q_nominal_specify=off  Q_nominal_unit=W  Q_nominal_value=1
      settings: SourceProductName=Simscape  SourceProductBaseCode=SS
  R_toWC_a(5) : fl_lib/Thermal/Thermal Elements/Thermal Resistance  resistance=R_toWC_a K/W  T_specify=off  T_priority=None  T=0 K  T_nominal_specify=off  T_nominal_unit=K  T_nominal_value=1  Q_specify=off  Q_priority=None  Q=0 W  Q_nominal_specify=off  Q_nominal_unit=W  Q_nominal_value=1
      settings: SourceProductName=Simscape  SourceProductBaseCode=SS
  R_toWC_p(1) : fl_lib/Thermal/Thermal Elements/Thermal Resistance  resistance=R_toWC_p K/W  T_specify=off  T_priority=None  T=0 K  T_nominal_specify=off  T_nominal_unit=K  T_nominal_value=1  Q_specify=off  Q_priority=None  Q=0 W  Q_nominal_specify=off  Q_nominal_unit=W  Q_nominal_value=1
      settings: SourceProductName=Simscape  SourceProductBaseCode=SS
  R_toWC_p(2) : fl_lib/Thermal/Thermal Elements/Thermal Resistance  resistance=R_toWC_p K/W  T_specify=off  T_priority=None  T=0 K  T_nominal_specify=off  T_nominal_unit=K  T_nominal_value=1  Q_specify=off  Q_priority=None  Q=0 W  Q_nominal_specify=off  Q_nominal_unit=W  Q_nominal_value=1
      settings: SourceProductName=Simscape  SourceProductBaseCode=SS
  R_toWH(1.1) : fl_lib/Thermal/Thermal Elements/Thermal Resistance  resistance=R_toWH K/W  T_specify=off  T_priority=None  T=0 K  T_nominal_specify=off  T_nominal_unit=K  T_nominal_value=1  Q_specify=off  Q_priority=None  Q=0 W  Q_nominal_specify=off  Q_nominal_unit=W  Q_nominal_value=1
      settings: SourceProductName=Simscape  SourceProductBaseCode=SS
  R_toWH(1.2) : fl_lib/Thermal/Thermal Elements/Thermal Resistance  resistance=R_toWH K/W  T_specify=off  T_priority=None  T=0 K  T_nominal_specify=off  T_nominal_unit=K  T_nominal_value=1  Q_specify=off  Q_priority=None  Q=0 W  Q_nominal_specify=off  Q_nominal_unit=W  Q_nominal_value=1
      settings: SourceProductName=Simscape  SourceProductBaseCode=SS
  R_toWH(2.1) : fl_lib/Thermal/Thermal Elements/Thermal Resistance  resistance=R_toWH K/W  T_specify=off  T_priority=None  T=0 K  T_nominal_specify=off  T_nominal_unit=K  T_nominal_value=1  Q_specify=off  Q_priority=None  Q=0 W  Q_nominal_specify=off  Q_nominal_unit=W  Q_nominal_value=1
      settings: SourceProductName=Simscape  SourceProductBaseCode=SS
  R_toWH(2.2) : fl_lib/Thermal/Thermal Elements/Thermal Resistance  resistance=R_toWH K/W  T_specify=off  T_priority=None  T=0 K  T_nominal_specify=off  T_nominal_unit=K  T_nominal_value=1  Q_specify=off  Q_priority=None  Q=0 W  Q_nominal_specify=off  Q_nominal_unit=W  Q_nominal_value=1
      settings: SourceProductName=Simscape  SourceProductBaseCode=SS
  R_toWH(3.1) : fl_lib/Thermal/Thermal Elements/Thermal Resistance  resistance=R_toWH K/W  T_specify=off  T_priority=None  T=0 K  T_nominal_specify=off  T_nominal_unit=K  T_nominal_value=1  Q_specify=off  Q_priority=None  Q=0 W  Q_nominal_specify=off  Q_nominal_unit=W  Q_nominal_value=1
      settings: SourceProductName=Simscape  SourceProductBaseCode=SS
  R_toWH(3.2) : fl_lib/Thermal/Thermal Elements/Thermal Resistance  resistance=R_toWH K/W  T_specify=off  T_priority=None  T=0 K  T_nominal_specify=off  T_nominal_unit=K  T_nominal_value=1  Q_specify=off  Q_priority=None  Q=0 W  Q_nominal_specify=off  Q_nominal_unit=W  Q_nominal_value=1
      settings: SourceProductName=Simscape  SourceProductBaseCode=SS
  R_toWH(4.1) : fl_lib/Thermal/Thermal Elements/Thermal Resistance  resistance=R_toWH K/W  T_specify=off  T_priority=None  T=0 K  T_nominal_specify=off  T_nominal_unit=K  T_nominal_value=1  Q_specify=off  Q_priority=None  Q=0 W  Q_nominal_specify=off  Q_nominal_unit=W  Q_nominal_value=1
      settings: SourceProductName=Simscape  SourceProductBaseCode=SS
  R_toWH(4.2) : fl_lib/Thermal/Thermal Elements/Thermal Resistance  resistance=R_toWH K/W  T_specify=off  T_priority=None  T=0 K  T_nominal_specify=off  T_nominal_unit=K  T_nominal_value=1  Q_specify=off  Q_priority=None  Q=0 W  Q_nominal_specify=off  Q_nominal_unit=W  Q_nominal_value=1
      settings: SourceProductName=Simscape  SourceProductBaseCode=SS
  R_toWH(5.1) : fl_lib/Thermal/Thermal Elements/Thermal Resistance  resistance=R_toWH K/W  T_specify=off  T_priority=None  T=0 K  T_nominal_specify=off  T_nominal_unit=K  T_nominal_value=1  Q_specify=off  Q_priority=None  Q=0 W  Q_nominal_specify=off  Q_nominal_unit=W  Q_nominal_value=1
      settings: SourceProductName=Simscape  SourceProductBaseCode=SS
  R_toWH(5.2) : fl_lib/Thermal/Thermal Elements/Thermal Resistance  resistance=R_toWH K/W  T_specify=off  T_priority=None  T=0 K  T_nominal_specify=off  T_nominal_unit=K  T_nominal_value=1  Q_specify=off  Q_priority=None  Q=0 W  Q_nominal_specify=off  Q_nominal_unit=W  Q_nominal_value=1
      settings: SourceProductName=Simscape  SourceProductBaseCode=SS
  Simulink-PS Converter{1..47} (47 alike) : nesl_utility/Simulink-PS Converter  PhysicalDomain=network_engine_domain  SubClassName=ps_input  LeftPortType=input  RightPortType=output  PseudoPeriodic=off  Frequencies=[]  NoiseDistribution=none  NoiseParameters=[]  Unit=1  AffineConversion=off  FilteringAndDerivatives=provide  SimscapeFilterOrder=1  InputFilterTimeConstant=0.001  UdotUserProvided=0
  Solver Configuration : nesl_utility/Solver Configuration  PhysicalDomain=network_engine_domain  SubClassName=solver  LeftPortType=input  RightPortType=generic  Tones=[]  Harmonics=[]  SimulateNoise=off  Profile=off  UseLocalSampling=off  EnableSwitchedLinearOptims=on  FrequencyDomain=off  UseCCode=off  RelTol=0.001  AbsTol=1e-06  MinStep=1e-09  ToWorkspace=off  RevertToSquareIcSolve=off  NumHomotopyIterations=100  PhasorMode=off  PhasorModeNumHarmonics=1  DoDC=off  ResidualTolerance=1e-09  UseLocalSolver=on  LocalSolverChoice=NE_BACKWARD_EULER_ADVANCER  LocalSolverSampleTime=dt  DoFixedCost=on  MaxNonlinIter=3  MaxModeIter=2  LinearAlgebra=auto  EquationFormulation=NE_TIME_EF  DelaysMemoryBudget=1024  AutomaticFiltering=on  FilteringTimeConstant=0.001  PartitionStorageMethod=AS_NEEDED  PartitionMemoryBudget=1024  PartitionMethod=FAST
  Subsystem : Subsystem
      settings: OpenFcn=open_system('simscape')
      mask Display: disp(sprintf('Open Simscape\nLibrary'));
  Subsystem1 : Subsystem
      settings: OpenFcn=|
      | load_system('fl_lib');
      | open_system('fl_lib/Thermal');
      mask Display: disp(sprintf('Open Thermal\nLibrary'));
  Switch : Switch  Threshold=pump_start_limit
  Switch1 : Switch  Threshold=pump_start_limit
  T_AGP(1) : fl_lib/Thermal/Thermal Sensors/Temperature Sensor
  T_AGP(2) : fl_lib/Thermal/Thermal Sensors/Temperature Sensor
  T_AGP(3) : fl_lib/Thermal/Thermal Sensors/Temperature Sensor
  T_AGP(4) : fl_lib/Thermal/Thermal Sensors/Temperature Sensor
  T_AGP(5) : fl_lib/Thermal/Thermal Sensors/Temperature Sensor
  T_EC(1) : fl_lib/Thermal/Thermal Sensors/Temperature Sensor
  T_EC(2) : fl_lib/Thermal/Thermal Sensors/Temperature Sensor
  T_ER(1) : fl_lib/Thermal/Thermal Sensors/Temperature Sensor
  T_ER(2) : fl_lib/Thermal/Thermal Sensors/Temperature Sensor
  T_HO_a(1) : fl_lib/Thermal/Thermal Sensors/Temperature Sensor
  T_HO_a(2) : fl_lib/Thermal/Thermal Sensors/Temperature Sensor
  T_HO_a(3) : fl_lib/Thermal/Thermal Sensors/Temperature Sensor
  T_HO_a(4) : fl_lib/Thermal/Thermal Sensors/Temperature Sensor
  T_HO_a(5) : fl_lib/Thermal/Thermal Sensors/Temperature Sensor
  T_HO_p(1) : fl_lib/Thermal/Thermal Sensors/Temperature Sensor
  T_HO_p(2) : fl_lib/Thermal/Thermal Sensors/Temperature Sensor
  T_IA(1) : fl_lib/Thermal/Thermal Sensors/Temperature Sensor
  T_IA(2) : fl_lib/Thermal/Thermal Sensors/Temperature Sensor
  T_RSL(1) : fl_lib/Thermal/Thermal Sensors/Temperature Sensor
  T_RSL(2) : fl_lib/Thermal/Thermal Sensors/Temperature Sensor
  T_RSL(3) : fl_lib/Thermal/Thermal Sensors/Temperature Sensor
  T_RSL(4) : fl_lib/Thermal/Thermal Sensors/Temperature Sensor
  T_RSL(5) : fl_lib/Thermal/Thermal Sensors/Temperature Sensor
  T_RTO(1) : fl_lib/Thermal/Thermal Sensors/Temperature Sensor
  T_RTO(2) : fl_lib/Thermal/Thermal Sensors/Temperature Sensor
  T_RTO(3) : fl_lib/Thermal/Thermal Sensors/Temperature Sensor
  T_RTO(4) : fl_lib/Thermal/Thermal Sensors/Temperature Sensor
  T_RTO(5) : fl_lib/Thermal/Thermal Sensors/Temperature Sensor
  T_RYO(1) : fl_lib/Thermal/Thermal Sensors/Temperature Sensor
  T_RYO(2) : fl_lib/Thermal/Thermal Sensors/Temperature Sensor
  T_RYO(3) : fl_lib/Thermal/Thermal Sensors/Temperature Sensor
  T_RYO(4) : fl_lib/Thermal/Thermal Sensors/Temperature Sensor
  T_RYO(5) : fl_lib/Thermal/Thermal Sensors/Temperature Sensor
  T_SH_a(1) : fl_lib/Thermal/Thermal Sensors/Temperature Sensor
  T_SH_a(2) : fl_lib/Thermal/Thermal Sensors/Temperature Sensor
  T_SH_a(3) : fl_lib/Thermal/Thermal Sensors/Temperature Sensor
  T_SH_a(4) : fl_lib/Thermal/Thermal Sensors/Temperature Sensor
  T_SH_a(5) : fl_lib/Thermal/Thermal Sensors/Temperature Sensor
  T_SH_p(1) : fl_lib/Thermal/Thermal Sensors/Temperature Sensor
  T_SH_p(2) : fl_lib/Thermal/Thermal Sensors/Temperature Sensor
  T_SSL(1) : fl_lib/Thermal/Thermal Sensors/Temperature Sensor
  T_SSL(2) : fl_lib/Thermal/Thermal Sensors/Temperature Sensor
  T_SSL(3) : fl_lib/Thermal/Thermal Sensors/Temperature Sensor
  T_SSL(4) : fl_lib/Thermal/Thermal Sensors/Temperature Sensor
  T_SSL(5) : fl_lib/Thermal/Thermal Sensors/Temperature Sensor
  T_STO(1) : fl_lib/Thermal/Thermal Sensors/Temperature Sensor
  T_STO(2) : fl_lib/Thermal/Thermal Sensors/Temperature Sensor
  T_STO(3) : fl_lib/Thermal/Thermal Sensors/Temperature Sensor
  T_STO(4) : fl_lib/Thermal/Thermal Sensors/Temperature Sensor
  T_STO(5) : fl_lib/Thermal/Thermal Sensors/Temperature Sensor
  T_SYO(1) : fl_lib/Thermal/Thermal Sensors/Temperature Sensor
  T_SYO(2) : fl_lib/Thermal/Thermal Sensors/Temperature Sensor
  T_SYO(3) : fl_lib/Thermal/Thermal Sensors/Temperature Sensor
  T_SYO(4) : fl_lib/Thermal/Thermal Sensors/Temperature Sensor
  T_SYO(5) : fl_lib/Thermal/Thermal Sensors/Temperature Sensor
  T_WC : fl_lib/Thermal/Thermal Sensors/Temperature Sensor
  T_WH(1) : fl_lib/Thermal/Thermal Sensors/Temperature Sensor
  T_WH(2) : fl_lib/Thermal/Thermal Sensors/Temperature Sensor
  Thermal Reference{1..103} (103 alike) : fl_lib/Thermal/Thermal Elements/Thermal Reference
  Umgebungslufttemperatur : fl_lib/Thermal/Thermal Sources/Temperature Source  temperature=T_Umgebung K
      settings: SourceProductName=Simscape
  Variable Thermal Resistance : fl_lib/Thermal/Thermal Elements/Variable Thermal Resistance  R_min=0 K/W  T_specify=off  T_priority=None  T=0 K  T_nominal_specify=off  T_nominal_unit=K  T_nominal_value=1  Q_specify=off  Q_priority=None  Q=0 W  Q_nominal_specify=off  Q_nominal_unit=W  Q_nominal_value=1
      settings: SourceProductName=Simscape  SourceProductBaseCode=SS
  Variable Thermal Resistance1 : fl_lib/Thermal/Thermal Elements/Variable Thermal Resistance  R_min=0 K/W  T_specify=off  T_priority=None  T=0 K  T_nominal_specify=off  T_nominal_unit=K  T_nominal_value=1  Q_specify=off  Q_priority=None  Q=0 W  Q_nominal_specify=off  Q_nominal_unit=W  Q_nominal_value=1
      settings: SourceProductName=Simscape  SourceProductBaseCode=SS
  air-gap convection AGP to RSL (1) : SimscapeCustomBlocks_lib/Convective Heat Transfer  area=A_RSL m^2  T_specify=off  T_priority=None  T=0 K  T_nominal_specify=off  T_nominal_unit=K  T_nominal_value=1  Q_specify=off  Q_priority=None  Q=0 W  Q_nominal_specify=off  Q_nominal_unit=W  Q_nominal_value=1
  air-gap convection AGP to RSL (2) : SimscapeCustomBlocks_lib/Convective Heat Transfer  area=A_RSL m^2  T_specify=off  T_priority=None  T=0 K  T_nominal_specify=off  T_nominal_unit=K  T_nominal_value=1  Q_specify=off  Q_priority=None  Q=0 W  Q_nominal_specify=off  Q_nominal_unit=W  Q_nominal_value=1
  air-gap convection AGP to RSL (3) : SimscapeCustomBlocks_lib/Convective Heat Transfer  area=A_RSL m^2  T_specify=off  T_priority=None  T=0 K  T_nominal_specify=off  T_nominal_unit=K  T_nominal_value=1  Q_specify=off  Q_priority=None  Q=0 W  Q_nominal_specify=off  Q_nominal_unit=W  Q_nominal_value=1
  air-gap convection AGP to RSL (4) : SimscapeCustomBlocks_lib/Convective Heat Transfer  area=A_RSL m^2  T_specify=off  T_priority=None  T=0 K  T_nominal_specify=off  T_nominal_unit=K  T_nominal_value=1  Q_specify=off  Q_priority=None  Q=0 W  Q_nominal_specify=off  Q_nominal_unit=W  Q_nominal_value=1
  air-gap convection AGP to RSL (5) : SimscapeCustomBlocks_lib/Convective Heat Transfer  area=A_RSL m^2  T_specify=off  T_priority=None  T=0 K  T_nominal_specify=off  T_nominal_unit=K  T_nominal_value=1  Q_specify=off  Q_priority=None  Q=0 W  Q_nominal_specify=off  Q_nominal_unit=W  Q_nominal_value=1
  air-gap convection AGP to RTO (1) : SimscapeCustomBlocks_lib/Convective Heat Transfer  area=A_RTO m^2  T_specify=off  T_priority=None  T=0 K  T_nominal_specify=off  T_nominal_unit=K  T_nominal_value=1  Q_specify=off  Q_priority=None  Q=0 W  Q_nominal_specify=off  Q_nominal_unit=W  Q_nominal_value=1
  air-gap convection AGP to RTO (2) : SimscapeCustomBlocks_lib/Convective Heat Transfer  area=A_RTO m^2  T_specify=off  T_priority=None  T=0 K  T_nominal_specify=off  T_nominal_unit=K  T_nominal_value=1  Q_specify=off  Q_priority=None  Q=0 W  Q_nominal_specify=off  Q_nominal_unit=W  Q_nominal_value=1
  air-gap convection AGP to RTO (3) : SimscapeCustomBlocks_lib/Convective Heat Transfer  area=A_RTO m^2  T_specify=off  T_priority=None  T=0 K  T_nominal_specify=off  T_nominal_unit=K  T_nominal_value=1  Q_specify=off  Q_priority=None  Q=0 W  Q_nominal_specify=off  Q_nominal_unit=W  Q_nominal_value=1
  air-gap convection AGP to RTO (4) : SimscapeCustomBlocks_lib/Convective Heat Transfer  area=A_RTO m^2  T_specify=off  T_priority=None  T=0 K  T_nominal_specify=off  T_nominal_unit=K  T_nominal_value=1  Q_specify=off  Q_priority=None  Q=0 W  Q_nominal_specify=off  Q_nominal_unit=W  Q_nominal_value=1
  air-gap convection AGP to RTO (5) : SimscapeCustomBlocks_lib/Convective Heat Transfer  area=A_RTO m^2  T_specify=off  T_priority=None  T=0 K  T_nominal_specify=off  T_nominal_unit=K  T_nominal_value=1  Q_specify=off  Q_priority=None  Q=0 W  Q_nominal_specify=off  Q_nominal_unit=W  Q_nominal_value=1
  air-gap convection AGP to SSL (1) : SimscapeCustomBlocks_lib/Convective Heat Transfer  area=A_SSL m^2  T_specify=off  T_priority=None  T=0 K  T_nominal_specify=off  T_nominal_unit=K  T_nominal_value=1  Q_specify=off  Q_priority=None  Q=0 W  Q_nominal_specify=off  Q_nominal_unit=W  Q_nominal_value=1
  air-gap convection AGP to SSL (2) : SimscapeCustomBlocks_lib/Convective Heat Transfer  area=A_SSL m^2  T_specify=off  T_priority=None  T=0 K  T_nominal_specify=off  T_nominal_unit=K  T_nominal_value=1  Q_specify=off  Q_priority=None  Q=0 W  Q_nominal_specify=off  Q_nominal_unit=W  Q_nominal_value=1
  air-gap convection AGP to SSL (3) : SimscapeCustomBlocks_lib/Convective Heat Transfer  area=A_SSL m^2  T_specify=off  T_priority=None  T=0 K  T_nominal_specify=off  T_nominal_unit=K  T_nominal_value=1  Q_specify=off  Q_priority=None  Q=0 W  Q_nominal_specify=off  Q_nominal_unit=W  Q_nominal_value=1
  air-gap convection AGP to SSL (4) : SimscapeCustomBlocks_lib/Convective Heat Transfer  area=A_SSL m^2  T_specify=off  T_priority=None  T=0 K  T_nominal_specify=off  T_nominal_unit=K  T_nominal_value=1  Q_specify=off  Q_priority=None  Q=0 W  Q_nominal_specify=off  Q_nominal_unit=W  Q_nominal_value=1
  air-gap convection AGP to SSL (5) : SimscapeCustomBlocks_lib/Convective Heat Transfer  area=A_SSL m^2  T_specify=off  T_priority=None  T=0 K  T_nominal_specify=off  T_nominal_unit=K  T_nominal_value=1  Q_specify=off  Q_priority=None  Q=0 W  Q_nominal_specify=off  Q_nominal_unit=W  Q_nominal_value=1
  air-gap convection AGP to STO (1) : SimscapeCustomBlocks_lib/Convective Heat Transfer  area=A_STO m^2  T_specify=off  T_priority=None  T=0 K  T_nominal_specify=off  T_nominal_unit=K  T_nominal_value=1  Q_specify=off  Q_priority=None  Q=0 W  Q_nominal_specify=off  Q_nominal_unit=W  Q_nominal_value=1
  air-gap convection AGP to STO (2) : SimscapeCustomBlocks_lib/Convective Heat Transfer  area=A_STO m^2  T_specify=off  T_priority=None  T=0 K  T_nominal_specify=off  T_nominal_unit=K  T_nominal_value=1  Q_specify=off  Q_priority=None  Q=0 W  Q_nominal_specify=off  Q_nominal_unit=W  Q_nominal_value=1
  air-gap convection AGP to STO (3) : SimscapeCustomBlocks_lib/Convective Heat Transfer  area=A_STO m^2  T_specify=off  T_priority=None  T=0 K  T_nominal_specify=off  T_nominal_unit=K  T_nominal_value=1  Q_specify=off  Q_priority=None  Q=0 W  Q_nominal_specify=off  Q_nominal_unit=W  Q_nominal_value=1
  air-gap convection AGP to STO (4) : SimscapeCustomBlocks_lib/Convective Heat Transfer  area=A_STO m^2  T_specify=off  T_priority=None  T=0 K  T_nominal_specify=off  T_nominal_unit=K  T_nominal_value=1  Q_specify=off  Q_priority=None  Q=0 W  Q_nominal_specify=off  Q_nominal_unit=W  Q_nominal_value=1
  air-gap convection AGP to STO (5) : SimscapeCustomBlocks_lib/Convective Heat Transfer  area=A_STO m^2  T_specify=off  T_priority=None  T=0 K  T_nominal_specify=off  T_nominal_unit=K  T_nominal_value=1  Q_specify=off  Q_priority=None  Q=0 W  Q_nominal_specify=off  Q_nominal_unit=W  Q_nominal_value=1
  inner air convection EC to inner air (1) : SimscapeCustomBlocks_lib/Convective Heat Transfer  area=A_EC m^2  T_specify=off  T_priority=None  T=0 K  T_nominal_specify=off  T_nominal_unit=K  T_nominal_value=1  Q_specify=off  Q_priority=None  Q=0 W  Q_nominal_specify=off  Q_nominal_unit=W  Q_nominal_value=1
  inner air convection EC to inner air (2) : SimscapeCustomBlocks_lib/Convective Heat Transfer  area=A_EC m^2  T_specify=off  T_priority=None  T=0 K  T_nominal_specify=off  T_nominal_unit=K  T_nominal_value=1  Q_specify=off  Q_priority=None  Q=0 W  Q_nominal_specify=off  Q_nominal_unit=W  Q_nominal_value=1
  inner air convection ER to inner air (1.1) : SimscapeCustomBlocks_lib/Convective Heat Transfer  area=A_ER_axial m^2  T_specify=off  T_priority=None  T=0 K  T_nominal_specify=off  T_nominal_unit=K  T_nominal_value=1  Q_specify=off  Q_priority=None  Q=0 W  Q_nominal_specify=off  Q_nominal_unit=W  Q_nominal_value=1
  inner air convection ER to inner air (1.2) : SimscapeCustomBlocks_lib/Convective Heat Transfer  area=A_ER_tang_i m^2  T_specify=off  T_priority=None  T=0 K  T_nominal_specify=off  T_nominal_unit=K  T_nominal_value=1  Q_specify=off  Q_priority=None  Q=0 W  Q_nominal_specify=off  Q_nominal_unit=W  Q_nominal_value=1
  inner air convection ER to inner air (1.3) : SimscapeCustomBlocks_lib/Convective Heat Transfer  area=A_ER_tang_a m^2  T_specify=off  T_priority=None  T=0 K  T_nominal_specify=off  T_nominal_unit=K  T_nominal_value=1  Q_specify=off  Q_priority=None  Q=0 W  Q_nominal_specify=off  Q_nominal_unit=W  Q_nominal_value=1
  inner air convection ER to inner air (2.1) : SimscapeCustomBlocks_lib/Convective Heat Transfer  area=A_ER_axial m^2  T_specify=off  T_priority=None  T=0 K  T_nominal_specify=off  T_nominal_unit=K  T_nominal_value=1  Q_specify=off  Q_priority=None  Q=0 W  Q_nominal_specify=off  Q_nominal_unit=W  Q_nominal_value=1
  inner air convection ER to inner air (2.2) : SimscapeCustomBlocks_lib/Convective Heat Transfer  area=A_ER_tang_i m^2  T_specify=off  T_priority=None  T=0 K  T_nominal_specify=off  T_nominal_unit=K  T_nominal_value=1  Q_specify=off  Q_priority=None  Q=0 W  Q_nominal_specify=off  Q_nominal_unit=W  Q_nominal_value=1
  inner air convection ER to inner air (2.3) : SimscapeCustomBlocks_lib/Convective Heat Transfer  area=A_ER_tang_a m^2  T_specify=off  T_priority=None  T=0 K  T_nominal_specify=off  T_nominal_unit=K  T_nominal_value=1  Q_specify=off  Q_priority=None  Q=0 W  Q_nominal_specify=off  Q_nominal_unit=W  Q_nominal_value=1
  inner air convection HO to inner air (1) : SimscapeCustomBlocks_lib/Convective Heat Transfer  area=A_HO2 m^2  T_specify=off  T_priority=None  T=0 K  T_nominal_specify=off  T_nominal_unit=K  T_nominal_value=1  Q_specify=off  Q_priority=None  Q=0 W  Q_nominal_specify=off  Q_nominal_unit=W  Q_nominal_value=1
  inner air convection HO to inner air (2) : SimscapeCustomBlocks_lib/Convective Heat Transfer  area=A_HO2 m^2  T_specify=off  T_priority=None  T=0 K  T_nominal_specify=off  T_nominal_unit=K  T_nominal_value=1  Q_specify=off  Q_priority=None  Q=0 W  Q_nominal_specify=off  Q_nominal_unit=W  Q_nominal_value=1
  inner air convection SH to inner air (1) : SimscapeCustomBlocks_lib/Convective Heat Transfer  area=A_SH m^2  T_specify=off  T_priority=None  T=0 K  T_nominal_specify=off  T_nominal_unit=K  T_nominal_value=1  Q_specify=off  Q_priority=None  Q=0 W  Q_nominal_specify=off  Q_nominal_unit=W  Q_nominal_value=1
  inner air convection SH to inner air (2) : SimscapeCustomBlocks_lib/Convective Heat Transfer  area=A_SH m^2  T_specify=off  T_priority=None  T=0 K  T_nominal_specify=off  T_nominal_unit=K  T_nominal_value=1  Q_specify=off  Q_priority=None  Q=0 W  Q_nominal_specify=off  Q_nominal_unit=W  Q_nominal_value=1
  inner air convection WH to inner air (1.1) : SimscapeCustomBlocks_lib/Convective Heat Transfer  area=A_WH_axial m^2  T_specify=off  T_priority=None  T=0 K  T_nominal_specify=off  T_nominal_unit=K  T_nominal_value=1  Q_specify=off  Q_priority=None  Q=0 W  Q_nominal_specify=off  Q_nominal_unit=W  Q_nominal_value=1
  inner air convection WH to inner air (1.2) : SimscapeCustomBlocks_lib/Convective Heat Transfer  area=A_WH_tang_a m^2  T_specify=off  T_priority=None  T=0 K  T_nominal_specify=off  T_nominal_unit=K  T_nominal_value=1  Q_specify=off  Q_priority=None  Q=0 W  Q_nominal_specify=off  Q_nominal_unit=W  Q_nominal_value=1
  inner air convection WH to inner air (1.3) : SimscapeCustomBlocks_lib/Convective Heat Transfer  area=A_WH_tang_i m^2  T_specify=off  T_priority=None  T=0 K  T_nominal_specify=off  T_nominal_unit=K  T_nominal_value=1  Q_specify=off  Q_priority=None  Q=0 W  Q_nominal_specify=off  Q_nominal_unit=W  Q_nominal_value=1
  inner air convection WH to inner air (2.1) : SimscapeCustomBlocks_lib/Convective Heat Transfer  area=A_WH_axial m^2  T_specify=off  T_priority=None  T=0 K  T_nominal_specify=off  T_nominal_unit=K  T_nominal_value=1  Q_specify=off  Q_priority=None  Q=0 W  Q_nominal_specify=off  Q_nominal_unit=W  Q_nominal_value=1
  inner air convection WH to inner air (2.2) : SimscapeCustomBlocks_lib/Convective Heat Transfer  area=A_WH_tang_a m^2  T_specify=off  T_priority=None  T=0 K  T_nominal_specify=off  T_nominal_unit=K  T_nominal_value=1  Q_specify=off  Q_priority=None  Q=0 W  Q_nominal_specify=off  Q_nominal_unit=W  Q_nominal_value=1
  inner air convection WH to inner air (2.3) : SimscapeCustomBlocks_lib/Convective Heat Transfer  area=A_WH_tang_i m^2  T_specify=off  T_priority=None  T=0 K  T_nominal_specify=off  T_nominal_unit=K  T_nominal_value=1  Q_specify=off  Q_priority=None  Q=0 W  Q_nominal_specify=off  Q_nominal_unit=W  Q_nominal_value=1
  pump active : Constant  Value=0
  pump inactive : Constant  Value=1000
  share of add losses in iron : Gain  Gain=0.5
  share of add losses in winding : Gain  Gain=0.5
  T_EMaschine_WH [K] : Outport
  T_EMaschine_Kuehlmittel [K] : Outport  Port=2
  T_EMaschine_SSL [K] : Outport  Port=3
  T_EMaschine_ER [K] : Outport  Port=4
  P_EMaschine_Verlust_ist [W] : Outport  Port=5
  T_EMaschine_STO [K] : Outport  Port=6
  T_EMaschine_AGP [K] : Outport  Port=7
  T_EMaschine_SYO [K] : Outport  Port=8
  T_EMaschine_RSL [K] : Outport  Port=9
  T_EMaschine_RTO [K] : Outport  Port=10
  T_EMaschine_RYO [K] : Outport  Port=11
  T_EMaschine_IA [K] : Outport  Port=12
  T_EMaschine_SH [K] : Outport  Port=13
  T_EMaschine_HO [K] : Outport  Port=14
  T_EMaschine_EC [K] : Outport  Port=15
  wires:
  HTC_Luftspalt [W*m^-2*K^-1]/1 -> Simulink-PS Converter6/1
  P_EMaschine_Verlust_Lager [W]/1 -> Gain4/1, Add/11  "P_EMaschine_Verlust_Lager [W]"
  P_EMaschine_Verlust_WirkZus [W]/1 -> share of add losses in winding/1, share of add losses in iron/1
  PS-Simulink Converter1/1 -> Bus Creator8/1  "T_EMaschine_WH_2 [K]"
  PS-Simulink Converter4/1 -> T_EMaschine_Kuehlmittel [K]/1  "T_EMaschine_Kuehlmittel [K]"
  HTC with coolant pump active/1 -> Switch/1
  HTC with coolant pump inactive/1 -> Switch/3
  Switch/1 -> Simulink-PS Converter4/1
  pump active/1 -> Switch1/1
  pump inactive/1 -> Switch1/3
  Switch1/1 -> Simulink-PS Converter3/1
  PS-Simulink Converter5/1 -> Bus Creator9/2  "T_EMaschine_ER_2 [K]"
  P_EMaschine_Verlust_Wicklung [W]/1 -> Aufteilung Wicklungsverluste + Temperaturabhängiger ohmscher Widerstand/5(P_EMaschine_Verlust_Wicklung [W])
  share of add losses in winding/1 -> Aufteilung Wicklungsverluste + Temperaturabhängiger ohmscher Widerstand/6(WirkZus-Verluste in Wicklung [W])
  Add/1 -> P_EMaschine_Verlust_ist [W]/1  "P_EMaschine_Verlust_ist [W]"
  Delay/1 -> Switch/2, Switch1/2
  Aufteilung Wicklungsverluste + Temperaturabhängiger ohmscher Widerstand/1(P_EMaschine_Verlust_SSL [W]) -> Add/1  "P_EMaschine_Verlust_SSL [W]"
  Gain4/1 -> Simulink-PS Converter9/1, Simulink-PS Converter19/1
  P_EMaschine_Verlust_Lueftung [W]/1 -> Aufteilung + Temperaturabhängigkeit Lüftungsverluste/3(P_EMaschine_Verlust_Lueftung [W])
  PS-Simulink Converter15/1 -> Bus Creator/1  "T_EMaschine_RYO_1 [K]"
  PS-Simulink Converter14/1 -> Bus Creator/2  "T_EMaschine_RYO_2 [K]"
  PS-Simulink Converter13/1 -> Bus Creator/3  "T_EMaschine_RYO_3 [K]"
  PS-Simulink Converter12/1 -> Bus Creator/4  "T_EMaschine_RYO_4 [K]"
  PS-Simulink Converter11/1 -> Bus Creator/5  "T_EMaschine_RYO_5 [K]"
  PS-Simulink Converter20/1 -> Bus Creator1/1  "T_EMaschine_RTO_1 [K]"
  PS-Simulink Converter19/1 -> Bus Creator1/2  "T_EMaschine_RTO_2 [K]"
  PS-Simulink Converter18/1 -> Bus Creator1/3  "T_EMaschine_RTO_3 [K]"
  PS-Simulink Converter17/1 -> Bus Creator1/4  "T_EMaschine_RTO_4 [K]"
  PS-Simulink Converter16/1 -> Bus Creator1/5  "T_EMaschine_RTO_5 [K]"
  Aufteilung Wicklungsverluste + Temperaturabhängiger ohmscher Widerstand/5(P_EMaschine_Verlust_SSL_bus [W]) -> Bus Selector/1
  PS-Simulink Converter25/1 -> Bus Creator3/1  "T_EMaschine_RSL_1 [K]"
  PS-Simulink Converter24/1 -> Bus Creator3/2  "T_EMaschine_RSL_2 [K]"
  PS-Simulink Converter23/1 -> Bus Creator3/3  "T_EMaschine_RSL_3 [K]"
  PS-Simulink Converter22/1 -> Bus Creator3/4  "T_EMaschine_RSL_4 [K]"
  PS-Simulink Converter21/1 -> Bus Creator3/5  "T_EMaschine_RSL_5 [K]"
  PS-Simulink Converter26/1 -> Bus Creator9/1  "T_EMaschine_ER_1 [K]"
  PS-Simulink Converter30/1 -> Bus Creator4/1  "T_EMaschine_AGP_1 [K]"
  PS-Simulink Converter29/1 -> Bus Creator4/2  "T_EMaschine_AGP_2 [K]"
  PS-Simulink Converter28/1 -> Bus Creator4/3  "T_EMaschine_AGP_3 [K]"
  PS-Simulink Converter27/1 -> Bus Creator4/4  "T_EMaschine_AGP_4 [K]"
  PS-Simulink Converter6/1 -> Bus Creator4/5  "T_EMaschine_AGP_5 [K]"
  PS-Simulink Converter8/1 -> Bus Creator8/2  "T_EMaschine_WH_1 [K]"
  Bus Selector/5 -> Simulink-PS Converter1/1  "<P_EMaschine_Verlust_SSL_5 [W]>"
  Bus Selector/4 -> Simulink-PS Converter11/1  "<P_EMaschine_Verlust_SSL_4 [W]>"
  Bus Selector/3 -> Simulink-PS Converter10/1  "<P_EMaschine_Verlust_SSL_3 [W]>"
  Bus Selector/2 -> Simulink-PS Converter8/1  "<P_EMaschine_Verlust_SSL_2 [W]>"
  Bus Selector/1 -> Simulink-PS Converter7/1  "<P_EMaschine_Verlust_SSL_1 [W]>"
  PS-Simulink Converter34/1 -> Bus Creator5/1  "T_EMaschine_SSL_1 [K]"
  PS-Simulink Converter33/1 -> Bus Creator5/2  "T_EMaschine_SSL_2 [K]"
  PS-Simulink Converter32/1 -> Bus Creator5/3  "T_EMaschine_SSL_3 [K]"
  PS-Simulink Converter31/1 -> Bus Creator5/4  "T_EMaschine_SSL_4 [K]"
  PS-Simulink Converter35/1 -> Bus Creator5/5  "T_EMaschine_SSL_5 [K]"
  PS-Simulink Converter9/1 -> Bus Creator6/1  "T_EMaschine_STO_1 [K]"
  PS-Simulink Converter7/1 -> Bus Creator6/2  "T_EMaschine_STO_2 [K]"
  PS-Simulink Converter3/1 -> Bus Creator6/3  "T_EMaschine_STO_3 [K]"
  PS-Simulink Converter2/1 -> Bus Creator6/4  "T_EMaschine_STO_4 [K]"
  PS-Simulink Converter10/1 -> Bus Creator6/5  "T_EMaschine_STO_5 [K]"
  PS-Simulink Converter40/1 -> Bus Creator7/1  "T_EMaschine_SYO_1 [K]"
  PS-Simulink Converter39/1 -> Bus Creator7/2  "T_EMaschine_SYO_2 [K]"
  PS-Simulink Converter38/1 -> Bus Creator7/3  "T_EMaschine_SYO_3 [K]"
  PS-Simulink Converter37/1 -> Bus Creator7/4  "T_EMaschine_SYO_4 [K]"
  PS-Simulink Converter36/1 -> Bus Creator7/5  "T_EMaschine_SYO_5 [K]"
  Bus Creator5/1 -> T_EMaschine_SSL [K]/1, Aufteilung Wicklungsverluste + Temperaturabhängiger ohmscher Widerstand/1(T_EMaschine_SSL [K])  "T_EMaschine_SSL [K]"
  Bus Creator8/1 -> T_EMaschine_WH [K]/1, Aufteilung Wicklungsverluste + Temperaturabhängiger ohmscher Widerstand/2(T_EMaschine_WH [K]), Bus Selector1/1  "T_EMaschine_WH [K]"
  Bus Creator6/1 -> Aufteilung + Temperaturabhängigkeit Ummagnetisierungsverluste/4(T_EMaschine_STO [K]), T_EMaschine_STO [K]/1  "T_EMaschine_STO [K]"
  Bus Creator7/1 -> Aufteilung + Temperaturabhängigkeit Ummagnetisierungsverluste/3(T_EMaschine_SYO [K]), T_EMaschine_SYO [K]/1  "T_EMaschine_SYO [K]"
  Bus Creator9/1 -> T_EMaschine_ER [K]/1, Aufteilung Wicklungsverluste + Temperaturabhängiger ohmscher Widerstand/3(T_EMaschine_ER [K])  "T_EMaschine_ER [K]"
  Bus Creator3/1 -> T_EMaschine_RSL [K]/1, Aufteilung Wicklungsverluste + Temperaturabhängiger ohmscher Widerstand/4(T_EMaschine_RSL [K])  "T_EMaschine_RSL [K]"
  Bus Creator1/1 -> T_EMaschine_RTO [K]/1, Aufteilung + Temperaturabhängigkeit Ummagnetisierungsverluste/5(T_EMaschine_RTO [K])  "T_EMaschine_RTO [K]"
  Bus Creator/1 -> T_EMaschine_RYO [K]/1, Aufteilung + Temperaturabhängigkeit Ummagnetisierungsverluste/6(T_EMaschine_RYO [K])  "T_EMaschine_RYO [K]"
  Bus Selector1/1 -> MinMax/1  "<T_EMaschine_WH_2 [K]>"
  Bus Selector1/2 -> MinMax/2  "<T_EMaschine_WH_1 [K]>"
  MinMax/1 -> Delay/1
  Aufteilung Wicklungsverluste + Temperaturabhängiger ohmscher Widerstand/2(P_EMaschine_Verlust_WH [W]) -> Add/2  "P_EMaschine_Verlust_WH [W]"
  Bus Selector2/2 -> Simulink-PS Converter20/1  "<P_EMaschine_Verlust_WH_1 [W]>"
  Bus Selector2/1 -> Simulink-PS Converter5/1  "<P_EMaschine_Verlust_WH_2 [W]>"
  Aufteilung Wicklungsverluste + Temperaturabhängiger ohmscher Widerstand/7(P_EMaschine_Verlust_ER_bus [W]) -> Bus Selector3/1
  Bus Selector3/1 -> Simulink-PS Converter13/1  "<P_EMaschine_Verlust_ER_1 [W]>"
  Bus Selector3/2 -> Simulink-PS Converter14/1  "<P_EMaschine_Verlust_ER_2 [W]>"
  Aufteilung Wicklungsverluste + Temperaturabhängiger ohmscher Widerstand/8(P_EMaschine_Verlust_RSL_bus [W]) -> Bus Selector4/1
  Bus Selector4/1 -> Simulink-PS Converter18/1  "<P_EMaschine_Verlust_RSL_1 [W]>"
  Bus Selector4/2 -> Simulink-PS Converter38/1  "<P_EMaschine_Verlust_RSL_2 [W]>"
  Bus Selector4/3 -> Simulink-PS Converter39/1  "<P_EMaschine_Verlust_RSL_3 [W]>"
  Bus Selector4/4 -> Simulink-PS Converter40/1  "<P_EMaschine_Verlust_RSL_4 [W]>"
  Bus Selector4/5 -> Simulink-PS Converter41/1  "<P_EMaschine_Verlust_RSL_5 [W]>"
  Bus Creator4/1 -> T_EMaschine_AGP [K]/1, Aufteilung + Temperaturabhängigkeit Lüftungsverluste/4(T_EMaschine_AGP [K])  "T_EMaschine_AGP [K]"
  Bus Selector5/1 -> Simulink-PS Converter12/1  "<P_EMaschine_Verlust_AGP_1 [W]>"
  Bus Selector5/2 -> Simulink-PS Converter42/1  "<P_EMaschine_Verlust_AGP_2 [W]>"
  Bus Selector5/3 -> Simulink-PS Converter43/1  "<P_EMaschine_Verlust_AGP_3 [W]>"
  Bus Selector5/4 -> Simulink-PS Converter44/1  "<P_EMaschine_Verlust_AGP_4 [W]>"
  Bus Selector5/5 -> Simulink-PS Converter45/1  "<P_EMaschine_Verlust_AGP_5 [W]>"
  Aufteilung + Temperaturabhängigkeit Lüftungsverluste/1(P_EMaschine_Verlust_AGP [W]) -> Add/9  "P_EMaschine_Verlust_Luftwiderstand [W]"
  share of add losses in iron/1 -> Aufteilung + Temperaturabhängigkeit Ummagnetisierungsverluste/1(WirkZus-Verluste in Eisen [W])
  P_EMaschine_Verlust_Ummagnet [W]/1 -> Aufteilung + Temperaturabhängigkeit Ummagnetisierungsverluste/2(P_EMaschine_Verlust_Ummagnet [W])
  Aufteilung + Temperaturabhängigkeit Ummagnetisierungsverluste/1(P_EMaschine_Verlust_Ummagnet_SYO [W]) -> Add/5  "P_EMaschine_Verlust_Ummagnet_SYO [W]"
  Aufteilung + Temperaturabhängigkeit Ummagnetisierungsverluste/2(P_EMaschine_Verlust_Ummagnet_STO [W]) -> Add/6  "P_EMaschine_Verlust_Ummagnet_STO [W]"
  Aufteilung + Temperaturabhängigkeit Ummagnetisierungsverluste/3(P_EMaschine_Verlust_Ummagnet_RTO [W]) -> Add/7  "P_EMaschine_Verlust_Ummagnet_RTO [W]"
  Aufteilung + Temperaturabhängigkeit Ummagnetisierungsverluste/4(P_EMaschine_Verlust_Ummagnet_RYO [W]) -> Add/8  "P_EMaschine_Verlust_Ummagnet_RYO [W]"
  Bus Selector6/1 -> Simulink-PS Converter15/1  "<P_EMaschine_Verlust_STO_1 [W]>"
  Bus Selector6/2 -> Simulink-PS Converter21/1  "<P_EMaschine_Verlust_STO_2 [W]>"
  Bus Selector6/4 -> Simulink-PS Converter24/1  "<P_EMaschine_Verlust_STO_4 [W]>"
  Bus Selector6/3 -> Simulink-PS Converter23/1  "<P_EMaschine_Verlust_STO_3 [W]>"
  Bus Selector6/5 -> Simulink-PS Converter22/1  "<P_EMaschine_Verlust_STO_5 [W]>"
  Aufteilung + Temperaturabhängigkeit Ummagnetisierungsverluste/6(P_EMaschine_Verlust_Ummagnet_STO_bus [W]) -> Bus Selector6/1
  Bus Selector7/1 -> Simulink-PS Converter17/1  "<P_EMaschine_Verlust_SYO_1 [W]>"
  Bus Selector7/2 -> Simulink-PS Converter25/1  "<P_EMaschine_Verlust_SYO_2 [W]>"
  Bus Selector7/3 -> Simulink-PS Converter27/1  "<P_EMaschine_Verlust_SYO_3 [W]>"
  Bus Selector7/4 -> Simulink-PS Converter26/1  "<P_EMaschine_Verlust_SYO_4 [W]>"
  Bus Selector7/5 -> Simulink-PS Converter28/1  "<P_EMaschine_Verlust_SYO_5 [W]>"
  Aufteilung + Temperaturabhängigkeit Ummagnetisierungsverluste/5(P_EMaschine_Verlust_Ummagnet_SYO_bus [W]) -> Bus Selector7/1
  Bus Selector8/1 -> Simulink-PS Converter33/1  "<P_EMaschine_Verlust_RTO_1 [W]>"
  Bus Selector8/2 -> Simulink-PS Converter34/1  "<P_EMaschine_Verlust_RTO_2 [W]>"
  Bus Selector8/3 -> Simulink-PS Converter35/1  "<P_EMaschine_Verlust_RTO_3 [W]>"
  Bus Selector8/4 -> Simulink-PS Converter36/1  "<P_EMaschine_Verlust_RTO_4 [W]>"
  Bus Selector8/5 -> Simulink-PS Converter37/1  "<P_EMaschine_Verlust_RTO_5 [W]>"
  Aufteilung + Temperaturabhängigkeit Ummagnetisierungsverluste/7(P_EMaschine_Verlust_Ummagnet_RTO_bus [W]) -> Bus Selector8/1
  Bus Selector9/1 -> Simulink-PS Converter16/1  "<P_EMaschine_Verlust_RYO_1 [W]>"
  Bus Selector9/2 -> Simulink-PS Converter29/1  "<P_EMaschine_Verlust_RYO_2 [W]>"
  Bus Selector9/3 -> Simulink-PS Converter30/1  "<P_EMaschine_Verlust_RYO_3 [W]>"
  Bus Selector9/4 -> Simulink-PS Converter31/1  "<P_EMaschine_Verlust_RYO_4 [W]>"
  Bus Selector9/5 -> Simulink-PS Converter32/1  "<P_EMaschine_Verlust_RYO_5 [W]>"
  Aufteilung + Temperaturabhängigkeit Ummagnetisierungsverluste/8(P_EMaschine_Verlust_Ummagnet_RYO_bus [W]) -> Bus Selector9/1
  Aufteilung Wicklungsverluste + Temperaturabhängiger ohmscher Widerstand/6(P_EMaschine_Verlust_WH_bus [W]) -> Bus Selector2/1
  Aufteilung Wicklungsverluste + Temperaturabhängiger ohmscher Widerstand/3(P_EMaschine_Verlust_ER [W]) -> Add/3  "P_EMaschine_Verlust_ER [W]"
  Aufteilung Wicklungsverluste + Temperaturabhängiger ohmscher Widerstand/4(P_EMaschine_Verlust_RSL [W]) -> Add/4  "P_EMaschine_Verlust_RSL [W]"
  Aufteilung + Temperaturabhängigkeit Lüftungsverluste/3(P_EMaschine_Verlust_AGP_bus [W]) -> Bus Selector5/1
  PS-Simulink Converter41/1 -> Bus Creator2/1  "T_EMaschine_IA_2 [K]"
  PS-Simulink Converter42/1 -> Bus Creator2/2  "T_EMaschine_IA_1 [K]"
  Bus Creator2/1 -> Aufteilung + Temperaturabhängigkeit Lüftungsverluste/5(T_EMaschine_IA [K]), T_EMaschine_IA [K]/1  "T_EMaschine_IA [K]"
  Aufteilung + Temperaturabhängigkeit Lüftungsverluste/4(P_EMaschine_Verlust_IA_bus [W]) -> Bus Selector10/1
  Bus Selector10/1 -> Simulink-PS Converter47/1  "<P_EMaschine_Verlust_IA_2 [W]>"
  Bus Selector10/2 -> Simulink-PS Converter46/1  "<P_EMaschine_Verlust_IA_1 [W]>"
  Aufteilung + Temperaturabhängigkeit Lüftungsverluste/2(P_EMaschine_Verlust_IA [W]) -> Add/10  "P_EMaschine_Verlust_IA [W]"
  HTC_fconv_Luftspalt [W*m^-2*K^-1]/1 -> Aufteilung + Temperaturabhängigkeit Lüftungsverluste/1(HTC_fconv_Luftspalt [W*m^-2*K^-1])
  HTC_fconv_Innenluft [W*m^-2*K^-1]/1 -> Aufteilung + Temperaturabhängigkeit Lüftungsverluste/2(HTC_fconv_Innenluft [W*m^-2*K^-1])
  PS-Simulink Converter47/1 -> Bus Creator10/1  "T_EMaschine_SH_p_2 [K]"
  PS-Simulink Converter48/1 -> Bus Creator10/7  "T_EMaschine_SH_p_1 [K]"
  PS-Simulink Converter46/1 -> Bus Creator10/2  "T_EMaschine_SH_a_5 [K]"
  PS-Simulink Converter45/1 -> Bus Creator10/3  "T_EMaschine_SH_a_4 [K]"
  PS-Simulink Converter44/1 -> Bus Creator10/4  "T_EMaschine_SH_a_3 [K]"
  PS-Simulink Converter43/1 -> Bus Creator10/5  "T_EMaschine_SH_a_2 [K]"
  PS-Simulink Converter49/1 -> Bus Creator10/6  "T_EMaschine_SH_a_1 [K]"
  Bus Creator10/1 -> T_EMaschine_SH [K]/1  "T_EMaschine_SH [K]"
  PS-Simulink Converter54/1 -> Bus Creator11/1  "T_EMaschine_HO_p_1 [K]"
  PS-Simulink Converter53/1 -> Bus Creator11/2  "T_EMaschine_HO_a_1 [K]"
  PS-Simulink Converter52/1 -> Bus Creator11/3  "T_EMaschine_HO_a_2 [K]"
  PS-Simulink Converter51/1 -> Bus Creator11/4  "T_EMaschine_HO_a_3 [K]"
  PS-Simulink Converter50/1 -> Bus Creator11/5  "T_EMaschine_HO_a_4 [K]"
  PS-Simulink Converter56/1 -> Bus Creator11/6  "T_EMaschine_HO_a_5 [K]"
  PS-Simulink Converter55/1 -> Bus Creator11/7  "T_EMaschine_HO_p_2 [K]"
  Bus Creator11/1 -> T_EMaschine_HO [K]/1  "T_EMaschine_HO [K]"
  PS-Simulink Converter57/1 -> Bus Creator12/1  "T_EMaschine_EC_2 [K]"
  PS-Simulink Converter58/1 -> Bus Creator12/2  "T_EMaschine_EC_1 [K]"
  Bus Creator12/1 -> T_EMaschine_EC [K]/1  "T_EMaschine_EC [K]"
  HTC_Innenluft [W*m^-2*K^-1]/1 -> Simulink-PS Converter2/1
  connections:
  R_toSH(1)/LConn1 -- T_RYO(1)/LConn1 -- C_RYO(1)/LConn1 -- PV_RYO(1)/LConn1 -- R_toRSLTO(1)/RConn1
  Thermal Reference7/LConn1 -- PV_SYO(1)/RConn2
  PV_SYO(1)/LConn1 -- R_toSSLTO(1)/LConn1 -- R_toHO(1)/RConn1 -- T_SYO(1)/LConn1 -- C_SYO(1)/LConn1
  R_toSYO(1)/LConn1 -- R_toSSLTO(1)/RConn1 -- R_toSYO2(1)/LConn1
  PV_SSL(1)/LConn1 -- T_SSL(1)/LConn1 -- C_SSL(1)/LConn1 -- R_toWH(1.2)/LConn1 -- R_toWH(1.1)/RConn1 -- R_toSTO(1)/RConn1 -- R_toSYO(1)/RConn1 -- R_toSAGP(1)/LConn1
  PV_BR(2.2)/LConn1 -- R_contactBR(2)/RConn1 -- R_toBR_p(2.2)/RConn1
  air-gap convection AGP to STO (1)/RConn1 -- R_toSAGP2(1)/RConn1
  R_toRYO2(1)/LConn1 -- R_toRAGP2(1)/RConn1 -- R_toRSL2(1)/LConn1 -- T_RTO(1)/LConn1 -- PV_RTO(1)/LConn1 -- C_RTO(1)/LConn1
  Thermal Reference12/LConn1 -- PV_AGP(1)/RConn2
  Thermal Reference8/LConn1 -- PV_STO(1)/RConn2
  R_toRAGP(1)/LConn1 -- air-gap convection AGP to RSL (1)/RConn1
  R_toWC_a(1)/LConn1 -- Convection HO to coolant (2)/LConn1
  R_toRSL2(1)/RConn1 -- R_toRTO(1)/LConn1
  Thermal Reference1/LConn1 -- PV_SSL(1)/RConn2
  Thermal Reference11/LConn1 -- PV_BR(2.1)/RConn2
  PV_STO(1)/LConn1 -- T_STO(1)/LConn1 -- C_STO(1)/LConn1 -- R_toSYO2(1)/RConn1 -- R_toSAGP2(1)/LConn1 -- R_toSSL2(1)/LConn1
  air-gap convection AGP to SSL (3)/LConn1 -- air-gap convection AGP to RSL (3)/LConn1 -- T_AGP(3)/LConn1 -- air-gap convection AGP to RTO (3)/LConn1 -- air-gap convection AGP to STO (3)/LConn1 -- PV_AGP(3)/LConn1
  Thermal Reference10/LConn1 -- PV_RYO(1)/RConn2
  R_toSSL2(1)/RConn1 -- R_toSTO(1)/LConn1
  Thermal Reference3/LConn1 -- PV_WH(2)/RConn2
  air-gap convection AGP to SSL (1)/RConn1 -- R_toSAGP(1)/RConn1
  R_toRAGP2(1)/LConn1 -- air-gap convection AGP to RTO (1)/RConn1
  R_toRSLTO(1)/LConn1 -- R_toRYO(1)/RConn1 -- R_toRYO2(1)/RConn1
  Variable Thermal Resistance/LConn1 -- C_WC water cooling pump active/LConn1 -- Variable Thermal Resistance1/RConn1
  Umgebungslufttemperatur/LConn1 -- Konvektion Radiator an Umgebungsluft (keine Geschw.Abhängigkeit)/RConn1
  Thermal Reference2/LConn1 -- T_WC/RConn1
  T_WC/RConn2 -- PS-Simulink Converter4/LConn1
  Convection HO to coolant (2)/LConn2 -- Convection HO to coolant (7)/LConn2 -- Convection HO to coolant (6)/LConn2 -- Convection HO to coolant (5)/LConn2 -- Convection HO to coolant (4)/LConn2 -- Convection HO to coolant (3)/LConn2 -- Convection HO to coolant (1)/LConn2 -- Simulink-PS Converter4/RConn1
  Convection HO to coolant (3)/RConn1 -- Convection HO to coolant (4)/RConn1 -- Convection HO to coolant (6)/RConn1 -- Convection HO to coolant (7)/RConn1 -- T_WC/LConn1 -- Convection HO to coolant (5)/RConn1 -- Convection HO to coolant (2)/RConn1 -- Convection HO to coolant (1)/RConn1 -- C_WC water cooling/LConn1 -- Variable Thermal Resistance/RConn1
  Variable Thermal Resistance1/LConn2 -- Variable Thermal Resistance/LConn2 -- Simulink-PS Converter3/RConn1
  T_ER(2)/RConn1 -- Thermal Reference14/LConn1
  Thermal Reference15/LConn1 -- T_RSL(3)/RConn1
  Thermal Reference13/LConn1 -- T_SSL(3)/RConn1
  R_toWC_a(5)/LConn1 -- Convection HO to coolant (6)/LConn1
  R_toWC_a(2)/LConn1 -- Convection HO to coolant (3)/LConn1
  R_toWC_a(3)/LConn1 -- Convection HO to coolant (4)/LConn1
  R_toWC_a(4)/LConn1 -- Convection HO to coolant (5)/LConn1
  C_HO_a(5)/LConn1 -- R_toSYO3(5)/LConn1 -- T_HO_a(5)/LConn1 -- R_toWC_a(5)/RConn1 -- R_toEC_a(5.1)/RConn1 -- R_toEC_a(5.2)/LConn1
  R_toEC_a(4.2)/RConn1 -- R_toEC_a(5.1)/LConn1
  C_HO_a(4)/LConn1 -- T_HO_a(4)/LConn1 -- R_toWC_a(4)/RConn1 -- R_toEC_a(4.1)/RConn1 -- R_toEC_a(4.2)/LConn1 -- R_toSYO3(4)/LConn1
  R_toEC_a(3.2)/RConn1 -- R_toEC_a(4.1)/LConn1
  R_toEC_a(2.1)/LConn1 -- R_toEC_a(1.2)/RConn1
  R_toEC_a(3.1)/LConn1 -- R_toEC_a(2.2)/RConn1
  R_toSYO3(3)/LConn1 -- T_HO_a(3)/LConn1 -- R_toWC_a(3)/RConn1 -- R_toEC_a(3.1)/RConn1 -- R_toEC_a(3.2)/LConn1 -- C_HO_a(3)/LConn1
  R_toSYO3(2)/LConn1 -- C_HO_a(2)/LConn1 -- T_HO_a(2)/LConn1 -- R_toWC_a(2)/RConn1 -- R_toEC_a(2.1)/RConn1 -- R_toEC_a(2.2)/LConn1
  R_toSYO3(1)/LConn1 -- T_HO_a(1)/LConn1 -- R_toWC_a(1)/RConn1 -- R_toEC_a(1.2)/LConn1 -- R_toEC_a(1.1)/RConn1 -- C_HO_a(1)/LConn1
  R_toHO(3)/LConn1 -- R_contactHO (3)/RConn1
  R_toHO(4)/LConn1 -- R_contactHO (4)/RConn1
  PV_SYO(2)/LConn1 -- R_toSSLTO(2)/LConn1 -- R_toHO(2)/RConn1 -- T_SYO(2)/LConn1 -- C_SYO(2)/LConn1
  Thermal Reference16/LConn1 -- PV_SYO(2)/RConn2
  PV_SYO(3)/LConn1 -- R_toSSLTO(3)/LConn1 -- R_toHO(3)/RConn1 -- T_SYO(3)/LConn1 -- C_SYO(3)/LConn1
  Thermal Reference17/LConn1 -- PV_SYO(3)/RConn2
  PV_SYO(4)/LConn1 -- R_toSSLTO(4)/LConn1 -- R_toHO(4)/RConn1 -- T_SYO(4)/LConn1 -- C_SYO(4)/LConn1
  Thermal Reference18/LConn1 -- PV_SYO(4)/RConn2
  PV_SYO(5)/LConn1 -- R_toSSLTO(5)/LConn1 -- R_toHO(5)/RConn1 -- T_SYO(5)/LConn1 -- C_SYO(5)/LConn1
  Thermal Reference19/LConn1 -- PV_SYO(5)/RConn2
  C_STO(2)/LConn1 -- PV_STO(2)/LConn1 -- T_STO(2)/LConn1 -- R_toSYO2(2)/RConn1 -- R_toSAGP2(2)/LConn1 -- R_toSSL2(2)/LConn1
  R_toSAGP(2)/LConn1 -- R_toSTO(2)/RConn1 -- R_toWH(2.2)/LConn1 -- R_toWH(2.1)/RConn1 -- T_SSL(2)/LConn1 -- C_SSL(2)/LConn1 -- PV_SSL(2)/LConn1 -- R_toSYO(2)/RConn1
  R_toSYO(2)/LConn1 -- R_toSSLTO(2)/RConn1 -- R_toSYO2(2)/LConn1
  air-gap convection AGP to STO (2)/RConn1 -- R_toSAGP2(2)/RConn1
  air-gap convection AGP to SSL (2)/RConn1 -- R_toSAGP(2)/RConn1
  Thermal Reference21/LConn1 -- PV_STO(2)/RConn2
  R_toSSL2(2)/RConn1 -- R_toSTO(2)/LConn1
  Thermal Reference20/LConn1 -- PV_SSL(2)/RConn2
  C_STO(3)/LConn1 -- PV_STO(3)/LConn1 -- T_STO(3)/LConn1 -- R_toSSL2(3)/LConn1 -- R_toSYO2(3)/RConn1 -- R_toSAGP2(3)/LConn1
  R_toSAGP(3)/LConn1 -- R_toSTO(3)/RConn1 -- R_toWH(3.2)/LConn1 -- R_toWH(3.1)/RConn1 -- T_SSL(3)/LConn1 -- C_SSL(3)/LConn1 -- PV_SSL(3)/LConn1 -- R_toSYO(3)/RConn1
  R_toSYO2(3)/LConn1 -- R_toSSLTO(3)/RConn1 -- R_toSYO(3)/LConn1
  air-gap convection AGP to STO (3)/RConn1 -- R_toSAGP2(3)/RConn1
  air-gap convection AGP to SSL (3)/RConn1 -- R_toSAGP(3)/RConn1
  Thermal Reference23/LConn1 -- PV_STO(3)/RConn2
  R_toSSL2(3)/RConn1 -- R_toSTO(3)/LConn1
  Thermal Reference22/LConn1 -- PV_SSL(3)/RConn2
  C_STO(4)/LConn1 -- PV_STO(4)/LConn1 -- T_STO(4)/LConn1 -- R_toSYO2(4)/RConn1 -- R_toSAGP2(4)/LConn1 -- R_toSSL2(4)/LConn1
  R_toSAGP(4)/LConn1 -- R_toSTO(4)/RConn1 -- R_toWH(4.2)/LConn1 -- R_toWH(4.1)/RConn1 -- T_SSL(4)/LConn1 -- C_SSL(4)/LConn1 -- PV_SSL(4)/LConn1 -- R_toSYO(4)/RConn1
  R_toSYO(4)/LConn1 -- R_toSSLTO(4)/RConn1 -- R_toSYO2(4)/LConn1
  air-gap convection AGP to STO (4)/RConn1 -- R_toSAGP2(4)/RConn1
  air-gap convection AGP to SSL (4)/RConn1 -- R_toSAGP(4)/RConn1
  Thermal Reference25/LConn1 -- PV_STO(4)/RConn2
  R_toSSL2(4)/RConn1 -- R_toSTO(4)/LConn1
  Thermal Reference24/LConn1 -- PV_SSL(4)/RConn2
  PV_STO(5)/LConn1 -- T_STO(5)/LConn1 -- C_STO(5)/LConn1 -- R_toSYO2(5)/RConn1 -- R_toSAGP2(5)/LConn1 -- R_toSSL2(5)/LConn1
  R_toSAGP(5)/LConn1 -- R_toSTO(5)/RConn1 -- R_toWH(5.2)/LConn1 -- R_toWH(5.1)/RConn1 -- C_SSL(5)/LConn1 -- PV_SSL(5)/LConn1 -- T_SSL(5)/LConn1 -- R_toSYO(5)/RConn1
  R_toSYO(5)/LConn1 -- R_toSSLTO(5)/RConn1 -- R_toSYO2(5)/LConn1
  air-gap convection AGP to STO (5)/RConn1 -- R_toSAGP2(5)/RConn1
  air-gap convection AGP to SSL (5)/RConn1 -- R_toSAGP(5)/RConn1
  Thermal Reference27/LConn1 -- PV_STO(5)/RConn2
  R_toSSL2(5)/RConn1 -- R_toSTO(5)/LConn1
  Thermal Reference26/LConn1 -- PV_SSL(5)/RConn2
  R_toWH(5.1)/LConn1 -- R_toWH(4.2)/RConn1
  R_toWH(4.1)/LConn1 -- R_toWH(3.2)/RConn1
  R_toWH(3.1)/LConn1 -- R_toWH(2.2)/RConn1
  R_toWH(2.1)/LConn1 -- R_toWH(1.2)/RConn1
  R_toSSL(2.1)/LConn1 -- R_toWH(5.2)/RConn1
  Thermal Reference29/LConn1 -- PV_WH(1)/RConn2
  Thermal Reference28/LConn1 -- T_WH(2)/RConn1
  PS-Simulink Converter1/LConn1 -- T_WH(2)/RConn2
  C_RSL(1)/LConn1 -- T_RSL(1)/LConn1 -- PV_RSL(1)/LConn1 -- R_toER(1.2)/LConn1 -- R_toER(1.1)/RConn1 -- R_toRAGP(1)/RConn1 -- R_toRTO(1)/RConn1 -- R_toRYO(1)/LConn1
  Thermal Reference30/LConn1 -- PV_RSL(1)/RConn2
  Thermal Reference9/LConn1 -- PV_RTO(1)/RConn2
  R_toRTO(2)/RConn1 -- R_toRAGP(2)/RConn1 -- T_RSL(2)/LConn1 -- C_RSL(2)/LConn1 -- PV_RSL(2)/LConn1 -- R_toER(2.2)/LConn1 -- R_toER(2.1)/RConn1 -- R_toRYO(2)/LConn1
  C_RTO(2)/LConn1 -- T_RTO(2)/LConn1 -- PV_RTO(2)/LConn1 -- R_toRYO2(2)/LConn1 -- R_toRAGP2(2)/RConn1 -- R_toRSL2(2)/LConn1
  R_toRYO2(2)/RConn1 -- R_toRYO(2)/RConn1 -- R_toRSLTO(2)/LConn1
  R_toBR_a(2.2)/LConn1 -- T_SH_a(2)/LConn1 -- C_SH_a(2)/LConn1 -- R_toBR_a(2.1)/RConn1 -- R_toRYO3(2)/RConn1
  R_toRSLTO(2)/RConn1 -- T_RYO(2)/LConn1 -- C_RYO(2)/LConn1 -- R_toSH(2)/LConn1 -- PV_RYO(2)/LConn1
  R_toRSL2(2)/RConn1 -- R_toRTO(2)/LConn1
  Thermal Reference32/LConn1 -- PV_RSL(2)/RConn2
  Thermal Reference33/LConn1 -- PV_RTO(2)/RConn2
  R_toRAGP(2)/LConn1 -- air-gap convection AGP to RSL (2)/RConn1
  Thermal Reference31/LConn1 -- PV_RYO(2)/RConn2
  R_toRAGP2(2)/LConn1 -- air-gap convection AGP to RTO (2)/RConn1
  R_toRTO(3)/RConn1 -- R_toRAGP(3)/RConn1 -- T_RSL(3)/LConn1 -- C_RSL(3)/LConn1 -- PV_RSL(3)/LConn1 -- R_toER(3.2)/LConn1 -- R_toER(3.1)/RConn1 -- R_toRYO(3)/LConn1
  C_RTO(3)/LConn1 -- T_RTO(3)/LConn1 -- PV_RTO(3)/LConn1 -- R_toRYO2(3)/LConn1 -- R_toRAGP2(3)/RConn1 -- R_toRSL2(3)/LConn1
  R_toRYO2(3)/RConn1 -- R_toRYO(3)/RConn1 -- R_toRSLTO(3)/LConn1
  R_toRSLTO(3)/RConn1 -- T_RYO(3)/LConn1 -- C_RYO(3)/LConn1 -- R_toSH(3)/LConn1 -- PV_RYO(3)/LConn1
  R_toRSL2(3)/RConn1 -- R_toRTO(3)/LConn1
  Thermal Reference35/LConn1 -- PV_RSL(3)/RConn2
  Thermal Reference36/LConn1 -- PV_RTO(3)/RConn2
  R_toRAGP(3)/LConn1 -- air-gap convection AGP to RSL (3)/RConn1
  Thermal Reference34/LConn1 -- PV_RYO(3)/RConn2
  R_toRAGP2(3)/LConn1 -- air-gap convection AGP to RTO (3)/RConn1
  R_toRTO(4)/RConn1 -- R_toRAGP(4)/RConn1 -- T_RSL(4)/LConn1 -- C_RSL(4)/LConn1 -- PV_RSL(4)/LConn1 -- R_toER(4.2)/LConn1 -- R_toER(4.1)/RConn1 -- R_toRYO(4)/LConn1
  C_RTO(4)/LConn1 -- T_RTO(4)/LConn1 -- PV_RTO(4)/LConn1 -- R_toRYO2(4)/LConn1 -- R_toRAGP2(4)/RConn1 -- R_toRSL2(4)/LConn1
  R_toRYO2(4)/RConn1 -- R_toRYO(4)/RConn1 -- R_toRSLTO(4)/LConn1
  R_toBR_a(4.2)/LConn1 -- T_SH_a(4)/LConn1 -- C_SH_a(4)/LConn1 -- R_toBR_a(4.1)/RConn1 -- R_toRYO3(4)/RConn1
  R_toRSLTO(4)/RConn1 -- T_RYO(4)/LConn1 -- C_RYO(4)/LConn1 -- R_toSH(4)/LConn1 -- PV_RYO(4)/LConn1
  R_toRSL2(4)/RConn1 -- R_toRTO(4)/LConn1
  Thermal Reference38/LConn1 -- PV_RSL(4)/RConn2
  Thermal Reference39/LConn1 -- PV_RTO(4)/RConn2
  R_toRAGP(4)/LConn1 -- air-gap convection AGP to RSL (4)/RConn1
  Thermal Reference37/LConn1 -- PV_RYO(4)/RConn2
  R_toRAGP2(4)/LConn1 -- air-gap convection AGP to RTO (4)/RConn1
  R_toRTO(5)/RConn1 -- R_toRAGP(5)/RConn1 -- T_RSL(5)/LConn1 -- C_RSL(5)/LConn1 -- PV_RSL(5)/LConn1 -- R_toER(5.2)/LConn1 -- R_toER(5.1)/RConn1 -- R_toRYO(5)/LConn1
  C_RTO(5)/LConn1 -- T_RTO(5)/LConn1 -- PV_RTO(5)/LConn1 -- R_toRYO2(5)/LConn1 -- R_toRAGP2(5)/RConn1 -- R_toRSL2(5)/LConn1
  R_toRYO(5)/RConn1 -- R_toRYO2(5)/RConn1 -- R_toRSLTO(5)/LConn1
  R_toBR_a(5.2)/LConn1 -- T_SH_a(5)/LConn1 -- C_SH_a(5)/LConn1 -- R_toBR_a(5.1)/RConn1 -- R_toRYO3(5)/RConn1
  R_toRSLTO(5)/RConn1 -- T_RYO(5)/LConn1 -- C_RYO(5)/LConn1 -- R_toSH(5)/LConn1 -- PV_RYO(5)/LConn1
  R_toRSL2(5)/RConn1 -- R_toRTO(5)/LConn1
  Thermal Reference41/LConn1 -- PV_RSL(5)/RConn2
  Thermal Reference42/LConn1 -- PV_RTO(5)/RConn2
  R_toRAGP(5)/LConn1 -- air-gap convection AGP to RSL (5)/RConn1
  Thermal Reference40/LConn1 -- PV_RYO(5)/RConn2
  R_toRAGP2(5)/LConn1 -- air-gap convection AGP to RTO (5)/RConn1
  R_toER(2.1)/LConn1 -- R_toER(1.2)/RConn1
  R_toER(2.2)/RConn1 -- R_toER(3.1)/LConn1
  R_toER(3.2)/RConn1 -- R_toER(4.1)/LConn1
  R_toER(4.2)/RConn1 -- R_toER(5.1)/LConn1
